simulink model "Noa_Nofusion_angle"  (R2020b)
settings: Solver=FixedStepDiscrete  StartTime=0.0  StopTime=Inf  FixedStep=0.01  RelTol=1e-3
PostLoadFcn:
  | if any(exist('dsrtsu_mdlpostloadfcn', 'file') ~= 0), dsrtsu_mdlpostloadfcn('Execute', bdroot); end
InitFcn:
  | , if any(exist('rtifpga_mdlclblib', 'file') ~= 0), rtifpga_mdlclblib('Init', bdroot); end,
  | , if any(exist('dsmpb_private', 'file') ~= 0), dsmpb_private('dsmpb_mdlclblib', 'Init', bdroot); end,
undefined symbols (not defined in the file): ACC_TimeGap_DecSetSwt, ACC_TimeGap_IncSetSwt, AccelPedalPosn, AccelPedalPosnVldty, AccelPedlPosnDiagc, AccPedalOverride, ACU_ShiftInProgress, ADAS_Posn_CurLane, AESSwtReq, ALC_SwtReq, BrkPedalSts, CC_ACC_CANCEL_OFFSwt, CC_ACC_CRUISE_OFFSwt, CC_ACC_DecSetSpd_SetSwt, CC_ACC_IncSetSpd_ResuSwt, CC_ACCSwtErr, CharSpd_ms, CSA_NODE, CURRENT_GEAR, CurrentGearValid, DiscIntNeverNeededParam, DrvDoorSts, DrvSBR, DrvTrqReqOvld, ECMACCInterface, ECMRespACC, ELKSwtReq, EngLimpHomeSts, EngSpd, EngState, EngState_PHEV, EngTrqMaxActSpd, EngTrqMinAct, EPS_DrvInpTrqVal_HighReslolution, EPS_FailSts, EPS_LKATorqOvrlDlvd, EPS_LKATorqOvrlDlvdVld, EPS_LKATrqOvlDlvdSts, EPS_SteerMod, EPS_TrqSnsrSts, EQ4_APPINFO, EQ4_LA_ELEM, EQ4_LA_HDR, EQ4_LAP_ELEM, EQ4_LAP_HDR, EQ4_LH_ELEM, EQ4_LH_HDR, EQ4_LRE_ELEM, EQ4_LRE_HDR, ESS_PedSwtReq, ESS_VehSwtReq, FFogLmpSts_F_Pbox, FLWheelDriveDirection, FLWheelSpd, FrntWiprSwtSts, FrntWshrSwtSts, FRWheelDriveDirection, FRWheelSpd, HazardLmpSwtSts, HCU_AccelPedalPosn_Diag ... (+151)
libraries: simulink x138, dsmpblib x33, canfdmsglib x10
(part 1 of 17)
PreSaveFcn:
  | , if any(exist('dsmpb_private', 'file') ~= 0), dsmpb_private('dsmpb_mdlclblib', 'PreSave', bdroot); end,
CloseFcn:
  | , if any(exist('dsmpb_private', 'file') ~= 0), dsmpb_private('dsmpb_mdlclblib', 'Close', bdroot); end,
settings Model: DataDictionary=HWA_DDs.sldd  RTICANMMDATA=struct('GeneralSetupData',struct('modelroot','D:\ADAS_Store\Project\adas_project','generalsettings',struct('filesettings',struct('destfolder',struct('Name','RTICANMM_FILES','Check',1),'buildfolder',struct('Name','.','Check',1),'AbsDestfolder',struct('Name','D:\ADAS_Store\Project\adas_project\RTICANMM_FILES'),'AbsBuildfolder',struct('Name','D:\ADAS_Store\Project\adas_project'))),'options',struct('addpaths',1,'rmpaths',1,'addtrcexclusion',false,'cannavigator',struct('checkmonitoring',0),'show_usrtrc',0,'use_usrtrc',0),'advanced',struct('options',ones(1,100)),'MPSetup',{{}},'RTI',struct('Type','DSRT','Ver','4.4','Date','02-Nov-2020'),'modelname','Noa_Nofusion_angle','block','Noa_Nofusion_angle'))  DSRTSU_INTERNAL_RTIFPGA=170  DSMPB_ID_DATA={'108889',struct('BlockId','81ba8c02-39a0-4bf8-971e-fc8bc9e1d8b0','SignalIds',{{'e6dae809-112a-4cbc-98f9-354c12187ac1','31d2deb7-ef93-4695-993d-314bc5bcc843','62343d78-d15a-4a45-8693-ba2849e89479','c13156af-d15b-4771-8a29-b8e73d565fa8','cbe04a47-fa20-4770-9bbd-4a07b568eb2e','59e00f7c-c03d-4b80-a5ec-a7b536bc6272','3f246c43-0baf-4388-bea8-c24249e8d124','05e7c6b4-9822-4e1b-91fa-c2d47c80a9dc','3c91b297-0034-4136-9460-a9a71fb1b160','b0eda23f-b1b7-44f7-9430-f2199b0de4f6','d9349f60-73fd-4e07-90cc-b8a5cfade7d1','f893d12f-c8e5-49d5-ab09-89fc2cdbf4b7','b489956b-9fe5-4db2-8485-d07366cb4569','0fd99c70-4fef-4ffb-8340-8501f6b1f5e4','53dd6ff7-6c1a-46a1-9139-61ea4f9d24e0','93fe1b5e-8abc-49f2-ae51-04c114465812','9444d888-9a75-4226-ace5-9b052183c8c8','ce7a08f7-cc95-444b-9a6f-cd5054dc142c','683a3bb5-05b9-4d71-b570-d34d769ae407','6e290ea9-9348-4509-bbba-48e715a1ad64','385761be-a1f9-4d98-b926-1efaecbe94cf','77479779-8c39-4f5c-be4f-4246b8ca51ff','094c4e00-d8db-4561-82fa-1990a2a46c70','8fedcf21-59e1-4a11-b24b-5edc3eea11e5','de2ede37-26b1-45c0-988c-7281b852313f','ed4cfff0-74cb-4a5b-9058-099c9444dc97','d8a92eb8-77b2-47c6-a14b-19e5a6c1880a','bb80831f-ec06-46fe-9a60-525cce3db11c','089a9e8f-4e14-4d97-a75c-e18256b8f73e','116e4020-4c03-4eaa-a133-5105e1ad6c2c','5d390f2c-fbfa-4acc-8e45-8a78ede6d630','e0ea540d-a3ce-47e8-9630-4c2a7c2611e9','1338e80f-eb11-478f-b148-febac8b5f561','40cb9f5e-abe1-4c5a-91b1-6a21a87629f0','f68eb2ae-9d65-4ce4-8ae6-7911307f53aa','90ccc115-d294-448b-be51-2f0d4ed4df75','d061fb9a-9168-48d0-bfc4-e7fc980285e5','66fbeac1-5405-448b-aaf2-b3b4c802c6b3','18d32c7d-1106-4865-b268-b9839028e3ed','68ea3199-eee5-4804-a61b-b9492c15cc17','251bf7c6-0b5c-4442-bed5-124eaca4f0a3','5c44ff7b-7cde-47e3-997c-d7e4d571a688','a318a3ac-fb11-4e42-abce-b283a20da434','8ac8bf9e-cc00-4453-b1d3-1d8cb9e4d5f3','e889ec5a-b6bf-4115-bfb4-789ddcbb1b39','843277e1-c8e1-4956-bb5f-69810b3fca13','8015402b-cae2-47f5-b799-3258863f20da','967f47db-98cb-4b9d-8737-8d02120e8039','408e6371-4b24-4e9e-8575-3f5fd9116599','0add38a7-641b-41d0-9036-40ff81d44c7c','42c9e777-d5c1-4821-b220-ee42a71da039','1eccc895-bd9f-4c89-9169-915b3accee5d','c32a22ec-25cc-4381-9457-3401f3ef52f2','dadafd58-4047-4fbe-8c61-d0d4f2e948e4','33df5bd2-20b0-4ead-bd24-c6cd609c4787','a6ef951d-803f-431b-afeb-b8db87ab93f4','3d89e518-12b9-4d0d-90f2-936f61a4e4f2','f4fba2eb-28a8-4b3f-a3d3-e6a85bead6df','1bbb28d7-2fef-43d6-b55d-c5356e90e304','46c1d4d9-bf71-419d-bdfe-9c3255f570d2'}}),'112056',struct('BlockId','6913c789-035b-4c0b-bbc8-df30b7210019','SignalIds',{{'6e67b619-d0e1-4489-8e12-cbb641b6930f'}}),'112939',struct('BlockId','bd32a928-034f-4d93-abe8-55cc1037974b','SignalIds',{{'ed378323-8937-4e58-90a7-af861033d965'}}),'112945',struct('BlockId','c5ed9ac9-a557-4e9e-b1b2-178e2ab00d3a','SignalIds',{{'9bf7ab65-611a-4ce6-8553-94d5ebac5e02','125861c6-7b90-4e8d-a590-5d6d82b8a9a7','4aee84b7-a55c-4fa5-a4b0-5c93a3e16834','bd31e0e7-f9ed-4a3b-9100-c48940e83979','f56bb652-89fc-4dda-9d9a-1212207cf3a7','0e2341be-0c6f-46b5-93e3-ba9acd4843ed','91d7f4b2-8cda-4163-9f74-f5dfcbc91f25','b0e338de-3225-4d50-a22b-4e417233ad31'}}),'21535',struct('BlockId','2585067a-bea5-4000-9f4a-5d4a5318ba82','SignalIds',{{'61f4e782-3c5c-4d26-b38e-7ab3a332c17d'}}),'21547',struct('BlockId','85c6324c-04f2-4bb9-ae49-a2215b872cec','SignalIds',{{'0e3885c9-c264-45e6-aecd-762fe1b73c31','1baabd13-ee21-4652-b6d4-ec6abbd58849','7652d1e7-3cbe-41d8-a4c1-1dd8e2fc5cb9','7bbccffc-d9cf-471f-ab9a-2a8c4994da51','a802a3dd-5a68-49d5-873f-4e8d27fb760e'}}),'26900',struct('BlockId','c4f53095-7434-4139-be7d-a6809331959f','SignalIds',{{'daa0d7ec-f8c9-46fb-8b57-637f6db1364b','6b9c406c-00c5-4598-bbc7-09f21b6102e2','f500b1a5-0ce1-46bf-9e31-2456a376294c','36025600-2dac-46a1-aa45-8494d12b2b41','ef53cc46-8ba2-4a58-bf53-0f87942fb3de','aa030106-e465-4c79-b00e-eff259d242dd','78eea2a2-72c6-4500-b175-67cd22d16487','1c2bede2-8500-4539-b1cb-e0ab955ea810','10a968e6-fd01-446e-bfca-b73896cbeda6','89b054e4-6567-474a-a101-bb566c01b012','298b31ac-930b-4ec4-925d-86f99e03a871','2a5dd987-b795-4b42-98e4-8e4e541ea47a','183af005-0028-4aae-8a97-0fded965b013','e1c3b11f-1e55-421d-b1c5-035f3444791f','d773bac5-9a48-4d62-be27-c6d96c81982f','04b9c5af-52d6-4c58-9c78-c1c20705dd99','e1e41399-89af-461d-9139-724a4d7cf416','0d5a1764-fbd7-4c90-8796-3b694c1b6f3d','99595cc9-51a9-4762-9eaa-0287cd22b3d1','74982970-242a-459f-a626-09b1e996aab8','e671e317-8ad6-460f-a115-14bde9303d0e','6aba3e83-cce1-4f14-959f-1b3259b2219c','3c1f9a12-89aa-43c9-9263-ad736254725b','e9e09c38-1a3c-4db0-b8eb-afc41c15f7ae','7d67eb52-960f-4419-a7b8-b5b57287a7ce','13d4f68a-7df0-4cd5-96cd-74a942b01dfb','b6834f02-cf2e-4d0c-83e8-3f5fbd5b4e80','11661590-7352-4bab-a498-0526255a2208','7f683842-0121-44e1-ac4c-b8ee6cdd73dc','13607d16-4de6-4b14-8b9a-e3fa31395056','9d7b37ef-0bbc-4717-993d-2cf555115b85','9cdb844a-f57f-45fa-9e48-b4a1a4b4896b','d36d0705-fbbd-4a92-912d-3076a1fef339','f1064f2a-d7e9-4f1e-a640-9b2d88534320','c7acaad8-e629-4dc2-8e05-0c6a9ba8cd34','12523044-5a8d-4a8b-aff1-248d7e37c730','d6a98294-c583-489b-9ba8-57c74dc9e44b','a662749b-cb79-4e22-b746-fb2c743a06c1','f430f874-81df-464f-a7d3-30981e4f10a2','beebc79e-c796-4a43-8cae-d93d3757c9ef','45edb788-142d-4d5e-b6bb-3d5a239307d1','f11dc556-f569-4261-bd02-c87d51a35c06','9fdd9cc9-7219-4342-b284-af726a522230','30d94524-5be1-4cf4-ae3c-2fca7636de21','0a9cc0a3-0bac-4d2d-8fdd-7eaacc91cba7','515fd30d-b8a5-4bf9-afb8-efc29c139c1c','7e6ceb3c-7950-428d-ac4b-43dfc5d8e62a','9a0a1488-4d4f-4ee5-9c00-712f8d888565','437104cc-392f-443f-b249-3988251c6d1d','ffdcc33a-9507-4d93-b2af-a5bcbf332fcd','ec49087a-871e-417b-9f51-df684f8a506d','9c70bacf-569a-4b32-9a53-2a08a50f21e1','c02297f7-a9d1-4ad2-9a5e-4508cee9802d'}}),'27021',struct('BlockId','bdf40dee-effa-4f83-9fca-9a80da5144bc','SignalIds',{{'6c1ed526-1be2-4bbd-bcae-90132b9ce65e'}}),'92096',struct('BlockId','2626a49c-eafb-489e-9e25-3cc30e7f0f4b','SignalIds',{{'3d8ff92d-3a53-4791-a9fe-7d0ec83fe68b','57fe1359-b477-4052-8b42-8fea101ccbbe','7ab6ec8e-bb47-446d-9b63-efa3400f4bc0','aae3fe2c-9486-44ef-a174-ff35666d1ac3','2728f40e-e3bc-46dd-820c-09fc547a2cf4','97772696-4328-4ad9-a419-0b1a5b3b5793','ee295b70-1271-4646-9bfa-8df6089991a4','624522df-0b73-4097-be1b-483fbaec0508','da88715c-b735-4415-8099-7b8d0dbc153e','ff209cfc-a262-4f28-baaf-3a6db897a966','e492b0bd-e407-499e-a6ad-460a06daea81','24f4850d-92b1-412a-9afe-0ffa2b28ac6e','e62d0e3a-07cf-4f2f-aed5-4364b9f58ffd','a952210a-42a9-4b58-aa64-8d3d5d349e0f','4a7d5fb8-0f46-4176-813b-55afe5653e46','44439239-e225-44a6-ba08-400a080bd9d0','d9d40cf9-f368-4b60-a6a2-4bed2dde0f48','50613ba6-c87d-4614-bf70-f0dff690fed6','171e7712-0418-4998-90fb-cbbc9f6a25a3','d8d9e3e9-d156-4676-ae37-3284503a7c6f','70f23cb8-d3ac-430b-8269-5a073a7d408e','efe9449e-e772-485f-b06b-2486dfc19974','7c476018-eb97-49c3-a1cf-2bcf515b1ac0','8ec107d4-18de-481c-b547-a0727ab809a5','45accd66-167c-4db8-ab27-6523ea2eac45','02953ce1-6202-4abb-9238-8ced4a0d88da','dab9925b-7344-4ce9-8745-111b6e6cae7d','c76755d9-df78-4ade-a507-373d8308233f','5fe272f0-e37e-4cdb-be86-e2af3525fe24','5793162b-b485-4d01-a81d-f3a4bacb08e6','a8a40964-43cd-4989-95ed-855ea1943846','f7248f97-efe7-4f34-b16b-ac2ba47ee6ba','84c9528d-5a3d-46b5-954d-d578c4df8378','3524f1a0-9033-4392-b170-0db3a27e414e','b9c5b901-2ee0-4cc1-a573-c8f9972649a5','b8ef879d-b046-4200-9baa-8e8fcd89cfbb','20f476a7-cf03-4f2c-a2fb-85aa3b4d50a6','caf3ad97-2086-496d-aaf6-47e61d3c29b6','c7efd7b8-2c78-44da-ae3a-28429611f8dc','45aa4b4f-2eb9-4971-82dc-61f3e357c005','2ca95a23-55a3-463e-975c-13578ef7d1bd','62c9d3f0-5102-4467-8adf-cf0fe7aa516d','e686d2ad-bd77-4dc9-b165-65d6d19e2eb2','9f4da501-daf3-4c3b-98bb-e7c10ddff144','1f52e3ff-314d-4fd2-9f3b-2179e824ba31','2af83930-d728-441e-9e4f-34537c4a20f5','e8860b5b-8674-401b-b995-34d5e2206f38','9dc95bcf-a38c-46f4-ad2d-2620ccd6e28c','b11c0df1-c523-4f91-8153-b13c114b944a','8b19ff0c-f7e1-4ee8-9507-7bfef01e81b7','e8150809-c884-401c-91ca-691eab8713b8','67b8761a-57df-4479-a70d-848ee2300e71','e9f52eab-a319-400d-b795-24d107b9bb7f','b66e22d5-841c-424d-ab80-4f02e6ec04c3','3d9b6ecb-ddee-4913-9e3b-4244499aa60e','593c337f-f38d-4a78-add4-e57c457ea88a','fdb5510f-5603-4091-94d5-66791780d419','9911966d-5645-473e-80de-5d7e0f980f21','6f7c21f8-8e7d-4b72-bbc3-0e10cb05173c','3cf030b9-a9fc-4f36-b3cd-b0ea10075552','5e21e0e9-e6af-401b-b8dc-f153ff7859a5','2ead1bcd-f571-40d5-b1b7-984cf6275c5e','676f31e3-b6c7-47a0-ad43-b760f2ef7778','366bc5b9-34ae-4f7a-b39d-9bc22bff78ee','550b7788-b500-4a37-bf74-1cd332e45fca','ed532467-088f-4cc3-b99c-2be22cd1f55b','5fe4a452-4c8f-498c-9e74-056d5e5fcb6d','de61477b-8899-4695-931e-e6dc9dff6f17','f08850ad-85e6-45a2-8f86-9c970bf65da7','a50dc5a8-222d-4853-a56b-c4c5f2030a28','1e12c040-3fae-4e1f-b57c-aed15b50cb60','33b8c258-adac-4232-a5aa-7cbd27f89e64','30c60cb9-0158-4875-b17e-2201775d3ef4','0158b5ae-3f92-4d64-a3ad-bb7474bb3a6e','e690eac3-fa9c-4927-b989-add4c8060ad0','af05ab49-1078-4638-8a14-6509f6efd732','bf24c6f7-dce4-4516-aad7-4a8c032ae8af','81991912-ea4d-4e27-8e78-5b0c76654bbc','c7fb6541-eaf8-43b3-b2ca-d9d981ac7d0f','58b9113d-cd63-4934-97dc-b52c923767b2','96e7cb82-855f-4587-9d3a-d7c5bb8fee74','c554e833-9797-47e7-bf0e-8b9fad210e74','cd4d30c3-fee1-4580-82e8-4f0beb8ab679','5834d1fe-a2db-47bb-acf7-aaea5892158e','7cf871d0-24ee-4dd7-9c90-16f120070cdf','7dffb819-f00d-4891-8820-5398d5acf060','24b69ebc-7c8a-4c7f-a3a9-5e9f7c52673e','f2ec1d12-c3d8-4df9-9d1f-8c9d9cc284f2','5ab44027-dfa8-4291-8ee7-384f014795d5','0c446405-c1fb-45ec-8845-28063d3c79cc','01d340e6-0f15-4ad2-8525-35bf2aa956dd','204515fc-fbea-4f63-b894-eef527e6bd9d','e0dca325-cb84-4f09-b568-622b6d4ccf91','60797110-5ba2-41dd-9826-79bd67f11f65','6c59198a-d826-4935-9238-c719cd5105ec','5f61e17f-4507-42cd-aa76-6f1039e0b56f','590781bd-a45d-47f7-ac2d-8a76d193c4ca','06b5c281-2053-4949-b9c9-acb1373d506c','829bc97f-26da-4467-981e-44e81b1cf974','d244fbcc-aa84-45b9-a934-2d34beee6c10','c03a08f6-16fb-43b3-b945-8ea80b9c454a','78b58307-773d-4ad4-ac80-3c426eb6d4a8','25944f9f-e7bf-43f5-9f90-4698741facbf','d139a39e-d189-4e55-94a8-a2d8b1aa8d57','a22eff47-2099-483b-bba2-0f2b5f9cd86b','1590cad8-88cd-4028-af3c-d2f3d779d367','86f8be12-a4b9-4ecf-87fe-8b25adef1b13','44ad9a06-49ee-4a33-bb9a-53a876073052','544623b1-218d-4bef-9f32-24cd6382c500','56dd516b-8b28-49da-84e3-05e53df87f53','fbba60d8-75ce-4bba-a6b7-394aab10a38c','536ac807-a0ee-4cf9-8faa-3ea45ddef2f1','78655c66-d146-4cad-97de-3e0ecdd3a2f9','db33c394-c73b-4406-b43b-5dac604c1e78','28e623dc-2b5a-4d50-a8a2-c5277908705e','85751a1c-63bf-4f97-9d1f-adab5e2a19a8','810aac47-5472-4f25-b9e7-f9f905304e89','18687fb3-d36e-4bf4-8873-298926c4bbb6','68c8c97a-1822-40b1-813a-27642dfa48f1','48e55f21-58ec-45a9-b6f1-31ef51cd1bf0','4cc1ecec-4a9d-4339-8d09-837ffcc25a27','0eaf747f-be20-4679-8033-16d430a74668','71f1aad6-0a58-4bc9-97cf-f58e1d8a4d7a','a575f744-505c-46da-8164-3f27d1a01f29','88c346a3-1222-412d-8c82-18bb32cb94f6','9c4dda8e-2c36-4a68-a520-345222c759f8','9a64fe60-86ec-4c53-a8be-0c368dad4863','cb05c1d9-09d9-4691-be10-38ccfdb68f67','20a3bf7a-1982-4296-8e2d-403a73f32733','eb52f21b-ee1b-4288-a0f4-332dcf652d5e','f65cee83-56b8-45cb-8458-d0096cf4994e','bab032c3-1da4-4612-9dc5-aff2ca75e79d','5176ddc3-9445-4ad6-a31e-042e42e290e3','d10d9d92-94a2-4b5b-80b8-f11cd38c3a59','5691495f-3af5-4ca8-844a-29a1f4400004','7c53693e-f3f0-4fe8-a3a1-54ddaec8b4d9','fc96d5ff-d377-4bbf-a28e-3e6a6dea7dd5','1e98929b-e7af-476e-af77-181ade8e652a','db202cee-d525-49ce-a926-71f25cecfae0','f23ee0e6-90c4-4426-bba6-88df4a770310','27e0d418-cfbc-4f53-ad0d-eb138646fc32','e585dbd5-ed73-471e-b9f0-10ab4a80ee54','07204a56-ebfc-4e5b-9c6d-82f4c0129d6e','90822bc5-41f0-4928-ab6d-fac63b5813cc','46c69ce7-cc6e-49b3-ae8a-a82c548a48ef','7b6ffa78-10e5-4210-8134-880aa24d68f3','94c28e1c-015a-4654-92a5-445b6d750e09','fee0eecf-773e-4070-a917-a579c9a22070','35c0ef53-0794-4280-a40f-615abcf31fe1','2e7a2d6f-cc05-4e9e-b974-61ed38c5e3a2','c8a5d024-bc45-4303-aad5-443d5a088151','531f8683-421d-4c50-ac9d-75407f48093f','f5b45fea-f8e6-42cd-acd6-91eb016667d7','28910d08-4039-4b9c-8464-6b26316e2112','a2e4e76d-37b2-4ee5-89cb-2016e27c3a0f','e25a7e01-8980-419f-984a-184cbdcc3045','7caf7c64-cfc6-4577-91b2-7b0ae61a5b70','f14a134e-e223-41bb-8b67-368551a07fe6','850e7f72-971e-48f6-b743-5f389edc33f1','be231029-9743-4673-9108-ade630e37c12','e2c6fd4c-3723-40fd-80ef-771b8340b045','0419d3dd-643a-476c-a243-f1eaa6a780c3','a683725e-482b-405c-a89e-a97d565a6064','8a4e4ce0-eaf0-428d-bfb5-d3362f879d15','e8b44cc4-137f-4451-aa6c-b51e1d43f117','000c1bba-a30d-40c8-bbd1-d305027f6501','043d9aa3-06c5-4059-9f63-2f6a5b7f1351','3f1e1b05-cd4a-4187-be4a-bf0ed78c3c42','d5757a81-b479-4372-a289-125bab7eb450','a3fe406d-cafc-4714-bb45-dc188105481e','38c6a662-de1c-4f75-ba1f-03d816189bb2','9b388ea7-b241-4201-85d4-239a0b36b8b7','8447252c-5f40-42d8-97e7-58ce273fbb3b','afca203f-fb32-4c43-9256-651048cb904e','04418faa-346d-42e0-ba90-20a3a68eb760','2e4f26b9-fbb0-4565-b220-ef4bd4876878','3f5e17f8-1d4c-466f-9a78-91929891ff2a','84465d9b-1101-4a34-8139-fab9fc9cbf4f','0de2d0bf-9fa0-44d2-893c-bcb712810756','dff52e5c-f10c-4e45-aaee-e871f06641fb','f58df008-19df-4468-a02f-efcf04c20781','83fb9323-d1b9-4495-95e4-c27cc9781ecc','aa7a6970-ca01-473f-8a65-a664dd364882','15332edd-13b6-4e95-b55f-1ddf2e4310b3','349fbd14-9300-4ff8-828a-1d78de258286','d0fa0445-40a4-472a-8913-8ffe2b60f13d','ff00bbce-7e63-416b-9fdb-4ed606b1a647','5023b9ad-1d78-4877-8621-66c99cbf9033','831d24a3-d149-43f8-9d5b-5402989fb5bd','805c8c6e-14d4-4dec-ad85-2314cb821987','5eb82689-b93b-4494-86b4-5d80ab075d18','122caa9c-802e-4351-a0a9-ed314f74f62d','b758e3da-1b08-4627-95d8-4267f30be063','9a29bf84-d57e-43eb-b40e-d47ffb77341f','1d1dac37-4d36-47c7-9661-96a4fdedacdb','2f29f70b-9b09-4c4c-974d-0d5004e34c80','642c19cd-43be-482c-a9a4-a822b4bcee85','e1288f9c-444a-4c82-832c-12df2471b08d','4587c4ce-f20f-4063-b6cb-58b15651d415','20fe301b-8a8c-4ea5-9763-048fe2f63d67','050947ac-02b2-4c95-99c6-1ab11244084a','93fab8b6-c071-4a2f-bb64-4a0ccf61c80e','fa2d3185-53d3-4297-a3a0-a5a26bba4129','41f55103-b8d9-4268-9f4b-38a1c7a2e090','9131575f-1513-44c4-8e40-dcea1bdc2c34','0f6f99df-f496-4d71-89d5-9d3f90c03f66','0784ce9a-c36a-4a5a-8079-f53b5037dea5','dce24de1-3b73-42a1-8d7d-b9ccc29b5585','613e1a0c-6586-4f78-abf8-e712a4506a21','325f16a7-6461-4dd7-bcfa-d3307cc77cc0','a56cdef0-1577-4bbe-a286-9e472b92f1e2','69fe0482-a70a-45cb-abe6-38f6e9ce5682','a1349f06-44e3-4a56-bc28-57c886e1179a','b17595e0-ef28-4479-9f5d-200244451920','90e25904-45eb-47b6-9092-c7ea319011f0','7a69f69e-ad38-4652-a990-2f14a164b033','830bdcf8-6bb9-462f-ae29-93ef8a59ba0e','2c0f0daf-9967-4453-994b-4ac2b76a3fe9','f86d2f2b-5748-4976-9625-ab8d5fc01a44','c4d4b03f-4b49-4fd9-bfda-5580df38df97','805d6294-3f53-4ed7-beea-f7762331b702','1cdf3370-4712-4d44-af91-44d4946fa4da','8194d2ec-5f1e-48e1-b65f-28fc37a23c0a','fb58e5b8-5237-4940-88b2-272d03922783','ad6c4650-8134-4838-add4-c8bc474b4668','72eca40f-2206-4b85-8624-1b6ae42f537c','044e3b49-78a0-42cb-984c-e66dcd598d05','8efee970-1d6e-414c-8f03-27a1d76d5a0f','97d41cbb-8d5a-4a83-9ba7-185b7fe2ea08','d68f95fd-b8bf-4d01-af7a-b4fb6eaf29c2','303db2e9-fc92-48d7-9ecb-906f70e1f416','eed1e3b2-fe0c-4562-8b46-54d63f8a7be2','651a94c2-122d-43a0-8367-ba20cb93991a','aec85a4f-512d-4291-b810-978491f2380d','a1ec1e82-f988-4698-b178-4f40f74e89dd','24a65454-a01f-4027-9898-08fd81dc5b4c','9e32fb24-0ee1-4893-ab7e-c2ed85e083fa','0ef10c6e-1151-4395-8f2b-6039b664dddd','3a73158e-3018-4153-8ced-d8d0e52f7920','17cd7138-e8bd-4f08-a03f-4a6c28dd26b3','dc6fe649-0f9d-4473-a4cc-c67f096792bd','3ff2c654-08e6-4a2e-a2c0-f2ccca39bd9a','267fdbc9-0013-4378-abac-1a3bc2508325','8cdcbb97-c6af-44f5-a81a-fca93d548d85','01e47132-7cb7-4a8d-b3b9-4acb1b5ba713','8adc715e-501f-43e3-b0c0-daecd1c071a4','f0e897b1-8dba-478b-bea5-a1c344bcc182','5dcf6f94-8217-4b56-b241-d3a06ba668a1','548dc5fa-44b2-4cdc-8253-6ed94beb141f','9518475d-e0f2-43f1-9d95-d8dd24590394','0a818e29-04c3-4567-bc47-310dcaf3d1a6','4308728a-b992-47f6-8bc9-b6e3f15d305c','1c3d6196-d166-4677-9203-c0a470623360','593a4882-3d5b-49e9-913a-e4ae0053ed37','d041851e-159e-4808-8d9d-19afdea47f88','4e06a3b3-ac88-4829-8269-0227281a727c','fe6471fc-70f9-486a-bf1f-77fec6457f9e','99d3fa79-1be3-4227-bd24-6e9746d4143f','a242adca-2b2d-4c38-8b84-0e9f4200f46f','e0312b30-d87b-4033-8dc5-803a5afeea56','e0b2bf1f-6a31-446e-9a38-87510d2ee6d6','f3d1dad0-76bd-484a-9865-5d8a0acf70ed','90a56866-adad-483f-a6ba-78f4b2b96364','6ef1b725-24c5-45c2-97f7-e06ae2b54272','7ca65932-c1cc-4218-8b36-982bfce690ef','0abdaaa0-732c-4bad-97a5-d541d143fd51','4580bbaf-11f5-4cc3-bdc7-6ba801093fbc','ae10fa7c-a526-46f6-bc3e-748a89a638fb','52432646-2d18-4636-a478-5f06272abf7c','58e81fc3-1290-4d08-83f8-c00e55bc61a6','c00e220c-50ab-4f97-b452-eb2acb0b0a38','4172b606-5824-4d39-9648-2c7e0c22fb24','92d5bc23-8f61-4ccd-8057-7934b5207acb','b948222e-6ed8-420e-bd4e-ccdcab12feb6','fa6d2daa-a272-414e-a20e-acc675712022','9dea2d2d-8814-4ccc-bcae-b111e1d9e5aa','54a8cf29-9aff-4017-8f9e-428b696d1089','87f29953-f87c-4770-9e8d-b92682e69ee7','cd4429c2-46d8-460a-b491-30d9c09fc7e4','992b789f-633a-4c0a-af80-5b9957a64f4d','cd96e18c-3161-4947-923f-704f1673541e','462109fa-53f9-4130-97fa-2cdfcf16764e','53aa0027-9c38-44e2-9ff8-11d8417f8f40','ac09190a-e396-4807-9600-d9fc98987922','965915a3-49fe-4e02-ad50-727e3e372404','2ec764b5-b421-4acd-9aac-9a2d38a7756c','61309634-1525-41ac-b1e2-f3cd920aba8f','d9bedbfc-3228-44ec-bc52-2f20e8a4efef','7a3d64b4-ec3a-49a4-b5f7-080940d90220','bbd22767-c34a-4a65-bb76-b8380c69f21d','ad79eb07-af72-409e-bbb0-85bc82707581','5c1507c2-9c52-43e6-b66a-79c718379997','c0331f0e-3149-47a5-9c34-c7d018c92a10','8f2db1ba-a0c7-4209-b52f-8eccad69a858','84c6bedc-52c7-42a1-a0a1-b4a7542e9ed9','1f92b609-3585-4b61-b2db-778546bf6a8e','01d30e4f-cac8-4824-93af-2c1aac36bbee','1c89c759-8a54-4581-95ef-e26b3a733658','ee674abd-2a37-4259-9eb6-d9255888ef59','f7fd4cc2-8d76-486d-930a-33f5615b083c','dba21ca1-4bdf-4256-93a4-396ed9567692','08368ec1-99dc-4993-b504-6e534f95d426','f7c68234-5b90-495a-b707-1e65d1a8d37f','d1a3221f-32cd-4871-a58d-8f09c41f27f5','0112242c-0417-4ad5-b3c5-3a459f843b2f','1e04c133-d319-482b-9251-df40ea67b952','e3caa92a-8aff-4969-9a66-8be756e416b3','bff3988c-0f04-4c00-ab11-511fd2885bf3','eb697231-e7c2-4f0b-8d08-3e2dd3b4bc61','da7f149a-3bbc-485f-bd77-e8024b9ac6b5','1970c710-01b7-4869-b3e0-1e5614a42f80','0e4a3b2e-da26-4b6a-8a04-f0448d43dee5','2090db71-2e79-416a-84c7-84fa5edd820c','fbacf9d5-caaa-4636-8d61-3c4aae20c5a0','0b794907-2465-4a16-96ce-03a3661d0a4c','5cf6edbc-c458-4222-adbb-ab36ab37922f','898d3560-a168-4d57-8ac5-9a1b49d5fae9','12e577df-4cf7-409d-90ca-61f8b3b69628','bbeff121-ebcb-4857-baee-cb9df93a1440','8f5c9992-fa36-47b8-904c-3c94a866fc5d','d3a1621a-0840-4db2-a6a9-d52c32742f95','044da422-aaa4-41ac-912a-a3ecf9bc9e93','2e0d1720-d393-4143-a3fb-dffdd518f6e2','94f19e2c-045a-45ae-9028-0bef41785d82','6d2e69e8-ae80-431c-a1c7-5a3af749dfb2','b13f59ab-a9ef-4c45-8096-a05a1ba1529e','baf016bd-eabf-4cf5-9623-d2492a80ffe0','0402e472-2211-40e9-83b8-81f64b39a834','1c0669c5-6fcf-4aa4-995e-ee01de78ffaf','76ffe772-3164-4a14-82e8-01cb3e790ec0','66eafd35-c5a1-49c7-b27e-01f2742a6223','151e4f6b-af5e-48fb-b8c5-8d7e1c4d16e8','9ea734bc-2b42-48b6-bda6-4ee1e2c507a1','c43f4775-bfb4-44c7-99be-d8ae236b5fab','a5544eb4-9c5d-42bf-88b4-f3a8071c5f34','cbc81f1e-cc95-4993-a44f-b717fdca880d','6e780ba0-987f-4908-bc50-38a8338ba23a','2947cd37-7e3e-4b83-aa29-ebfadc627cd2','f0d78749-ec35-4fef-998e-a36372f4242f','19c1c3b9-9704-45dc-9ecf-153593b768af','9f4f3150-dce1-4cdc-a791-d27b79529b7c','ae2add4a-81b5-4ef5-98f5-458fa7c1dd7d','5551d896-095c-4cb8-8d58-f3cb1761b068','3f7f7b9a-0573-426d-823e-001a842fce79','e95db9d7-7856-4ebd-9a78-0010bfd540d9','fc8ca16c-c780-42a8-b649-447d66deff20','a8fd2a99-d6bc-4412-8ba1-d94bfa2126a0','e1a70efa-db41-4cfd-b40c-c01cf48262fe','728a0f41-4209-4dd0-b562-cf253b8fce54','bdd9150e-61ee-4bc6-8b3e-43c3253b1aab','f5a24cc0-9cfb-4fae-8fe2-74074a21b079','c6bce8fa-674d-4198-8f60-d6969c79a83a','f21c9b29-6525-48fb-9ecc-3680e67cd314','597c418f-3f02-46f2-930d-2eb9c8807c97','8307be91-76c8-4d78-b268-e765f17f8213','b296ac75-36a7-416d-8475-ffbe6e28dccd','894d960e-802e-4f7a-8988-49627d5ba1df','a63e3140-6046-42d5-8e51-0dd32a1f13b2','8b1e169e-5056-439a-bec1-36baa2e9bbe6','a4a3995f-113a-4dc4-b25a-be8bd1da7387','86db2c15-45a3-41bf-8c56-214272ed971f','381093e1-ab66-4e06-8fa4-4456f17711fd','076fb968-2186-4b91-ac30-2c432f9a9177','ab926246-8b0f-4aaa-9f36-675b3e24831c','1c642a3f-1918-46ff-ba78-fb9d552662c2','e2f89cdf-10b2-4393-96fc-de0fa61990cb','d6804f24-e5a9-4555-a6b1-6f9220e6faee','5b9b6444-8e5b-429a-ab3b-bd226f4f6762','00259496-7a4e-4736-88b0-c3b2f79e1a6c','ce5c8401-1f96-4f9f-aea1-45add305c888','4b72b3c2-128b-40ce-b5a5-e6203ab8306d','a6696863-16ac-41e6-bdf2-7a9e7e2f50c5','5579eb2c-854a-4fc6-b271-5eeb4e997a7e','1a658b2f-1574-49ce-b65a-4246003d54a0','74560410-1615-4c09-8363-96550de29c30','b0419aad-872c-4c24-add1-f2860d6fdcd9','e97708e4-c852-40a8-ae18-987509e18a13','8cff1538-1894-4d55-b669-06693e404479','b4ed3a7e-f2aa-40f9-b923-b562909472d0','c4175113-de5f-468b-be98-58087cc64d65','74c16fa2-c833-47bd-8b19-6877a026f3b7','5b0411c3-d5cb-4aef-a067-37da547447fe','61c5c432-b1c5-43ca-b42b-5d4e80c0df73','b1af5bfb-206e-4a56-8ec4-1474445a9bb0','f2af43f6-5b91-4976-9137-7ac836e13615','8c65d3c4-3cc0-42b7-a4fc-d34618147aae','bbeb1f63-8ec8-4a7a-aa7f-0a0670ba8c53','5e0b7212-de20-4b90-8167-a1d8d71b3581','7d6161bf-e6c5-42d4-9fb0-c855bf3c35ef','c01509f7-092e-4f93-8686-3d0b2ee8030a','aada585b-6d20-4d9d-b905-db9ebdcb35e9','7395536b-d0bd-403a-9077-1497efab2e29','8c2fee1d-b5f8-4c47-8b73-94a48fda8fa8','0c480f36-c97c-4ac8-a400-ee222e844362','16a2cd31-dec7-480d-8797-555f0d0a5951','f4a70afd-024d-4f0f-b108-98c72aefbd06','26a6634a-5557-42e2-951f-9ea525d513f6','3f0257f4-823e-42fc-ba1c-f70d652cdf0a','073b2b0e-cf48-45bc-bede-14afe0caa544','579a02fb-b4f5-4474-baa3-be64164def26','b0704ab8-8b9b-4f88-9a9b-873252207f84','9fb165fc-676b-47e8-9f44-531aeddf420c','12021c71-200f-432f-b9fd-2e69e6219535','1d7c976c-cdd2-4f7c-bad9-d2915e0485a7','f042261a-1bbc-4244-a964-2c8a0400aee3','5d1e84a2-3a42-48b8-a30b-c4b129cb754d','d2d41370-9876-4a7a-8de8-82f700e2f03c','90c2780e-80ef-4d54-98c7-24cdec16d72d','1aaa07be-19a6-4a4e-b6c4-511fa69433da','29bff75d-aea4-44ef-8dc7-dc2cdad6fd2e','22ba7138-1ce2-4c61-a335-28ded396f934','989b80e4-704a-4c79-903d-8ae53082e8b2','fdd8c6be-3c96-487f-8664-c518a8233547','35bca300-b763-439b-b9bf-23b09aac20d7','2878a9f4-83bf-4f74-970d-26ffd3d1caa8','19b50e68-db39-410f-beea-1741deb1b001','356c795f-fb51-43fe-bbf9-7030ffa63985','fd17d122-5e4d-4f7e-a9c9-a6d311502c23','6f549206-f745-4fbe-bf4a-5971d91758a2','52b171e1-cd33-41cb-b377-677409a7428b','551f39ec-44be-49ae-99f7-8fbb47c7fdcb','d8292ad8-043d-4ab8-948d-47cfa9b3b904','5468b3eb-6bb6-4413-81f8-489f4a61756b','94faf67a-fd83-4b87-be96-f76b816bf144','091e0108-cdd1-4850-bd0f-da47856ad13f','419c7e64-d721-4347-816b-01c998daa6af','46a4906e-9ba3-4399-aa15-7a1930adf60c','b1daf8f4-29ea-4d18-b082-e664e9f00a9b','eca1e40b-03b0-4193-9add-170578cd8756','f85399d2-b264-4259-9e9f-004db37898b6','c3d31f73-a62b-4485-b7bd-52724527d350','be9a7d52-5fd9-4b4c-9cac-84dbc16e868a','280d8570-faab-43ae-8673-e4770aca2299','c2f14551-2fa6-4f5d-9652-86ed23f67bb1','654f0f09-1430-4fe4-92ec-50ce00b1dc5f','b49b834c-ec9c-436f-88fa-7366e4573437','58f0fadd-680b-4055-86a2-d55f3f3f8f82','51325ea2-6a32-4c67-bb76-21573a2169b9','bc1c4ecb-3aa4-4f43-8caf-4662ecbe2eb9','53d1839b-9066-4927-9676-63bbcad37348','d0060f5d-6577-4748-b4b3-c8b6ce68a578','3d0fcec5-b4f6-4c22-8482-8ff5ed200b59','0ef00a85-d4c5-40c8-8637-dcf3d4564715','5deaf227-9f03-4762-9848-fd8ef131a10e','dd0833b3-03b1-4a69-82f2-76d1e8bc892c','eeb776f6-7b81-4219-836e-3f3be3cd9695','20c66184-f6c2-4d0e-bee4-31bd34f6057d','d851385a-e66d-48b7-a8bf-76b0714d7a68','f1077060-e81c-48ff-b9e6-e70828d15019','fd80642c-b57a-463a-b181-2be25a097bf8','a9ebf9d5-2f80-42e4-8e20-38bb855c96e6','4687720e-f564-49a4-9c3e-f036b574187f','ad1ca5d7-4b96-4096-8c8c-67aaba8eeec6','50f88368-7cb7-4366-97f5-c5c325e90273','b7c92691-c7d9-43bc-b69d-92b843ea7158','60c03145-284e-4852-ad84-286e71e9ea72','e4dd28a8-995c-4fca-b0c2-ec4f24e2424a','aac9f0fe-ef3e-4826-b52e-c15681203e9e','aba80fca-825b-4c99-8963-dc1ee96d5b4b','2e45b1df-cd50-4b76-ab31-6a45cf9ae826','988e9de7-e2cc-4c9a-b1af-0357ac723711','3974ac48-9636-46cd-b33f-a733d462f3cb','0e4c31bc-9b88-4444-9e87-80ca52fb743b','c517967b-e221-44b9-9af4-12bd06773eb4','175e145a-8343-4bf6-94b7-9391521a5986','a95faa5c-3511-401d-b485-deefaeac2792','4b78abc4-2c5f-46e6-85ed-1c48369341fa','5e1f4c94-6e78-4788-b6f4-0ce9a3b99af9','73960f8c-ca68-4dbf-9e53-53729829fa51','79c4c0c3-359f-4fae-bd0f-703e728dc7f4','c5ef383c-7477-4fbf-8f2a-8c34570b0a60','879407c9-45b1-4cb9-a337-93d3db86b180','082194e7-ed30-4db5-8633-7802f160bb72','946af0f8-9335-4e78-80ea-1d5e85c38cf8','4e6f7f2c-433f-4c8b-b57e-0223170cef3f','1879369c-4975-47d8-b161-b9458b2e2e0a','bf825221-13e7-46b7-8d8a-6bcd9cc70f45','6f4aac89-67e5-403e-8ea2-3e64eaecf5bf','7596f3bb-92db-4460-93a5-624b2e104dfe','299678b6-461f-4c28-96e0-8124d01cf03e','010a117f-131f-4284-9371-9989545410a5','e4c22902-2650-48ac-ba80-c23785a87932','afd4b235-6a4f-455d-a240-409af2e6d646','8ad1ef57-2671-4903-8b6d-55e96aab5b8d','8bc62295-df99-48d3-8281-dca323b41dc1','5f3503e6-9146-416a-b65a-715c87891207','a978b935-72e1-4a6a-a353-e8e80c7b2e60','76243153-fd90-42e4-8b0e-49392d590d6e','2d324350-e7d4-4d02-9509-0c033d157d98','c4130826-e813-4553-9ff6-fd150077a4e9','bce17a2b-86a6-4113-ae93-9ba9592fea9a','2e372e71-df2a-418b-99b5-e60dcae02d7d','5705a4d0-231a-4f76-a718-743fc7760f97','426cfcf9-cd7f-4c69-ac15-b1ecddbf17a8','f36e64a7-5c89-4d76-9010-d827432252be','fd3acf14-20e9-47e3-8df3-591469caca75','0a706e06-c899-42c3-8046-58b2d3fc7d91','f5b1242a-cdb0-4af8-8de0-89eda9ee4d9d','bdbb7bd3-fcd5-4dc7-b094-8b43f8065cfa','4a2c0b2b-7407-41d5-b28a-9dd2e33d491a','aa7fbad8-96a5-483f-8977-f1ba9f15b5d2','160fa7db-1b26-438b-9987-cdbec0a93ad4','0763ba0f-efde-43e7-8255-56e978c1629b','6f4a8351-045e-4a29-a9ee-9b93daa006a4','22597645-6d42-4252-a7e3-185db38ec2d2','1f38a729-2f1a-44fd-b72d-137b48266fa6','e2f52da7-f5f0-4baf-895b-3029a291ce3c','8c543016-e72c-40f6-96a4-336a89459910','e6dbaa1b-97ef-4f0d-9256-b9810fe718b1','e1780a4c-0559-42c0-aad4-480aa5ff3778','4279d1c3-c688-4fce-a8d7-2ae62dc9ca96','2c8f4d07-16aa-4577-91ae-76df51f10279','5563937b-4b16-4ce6-b827-117152b4a5ec','1c991fa4-1549-4d78-8288-b10e4ca2998b','0b6d48e7-3820-4fad-88c1-63ec63443a08','ebe2e4e7-e2f0-41d5-aa89-f785ccc8ec3a','38ae271c-c8d5-4a03-8013-9ec2c47529cd','0790e15a-6b8a-4845-9d21-328a736df5b4','d67511eb-f783-4f61-88ae-1490d2572145','d3bdd845-64a0-46b0-b476-dca13ced2ffc','b736b726-8c68-48ef-b37f-962bee919652','b9a7c64b-9f8d-4190-9f24-e2f792e11502','10a527cf-1826-4f5f-b5a3-4ca107957394','ad926b5a-bf53-4a24-bb33-d2f9205e9bc0','eb285f61-3d8a-4fe0-b4d0-39bbbb443f82','c4ec9191-8bc3-450f-9716-6f453cdd812a','832f16bc-c43f-423a-97b6-e3dac3bffdfc','47583840-8eef-4d12-8cc8-76d2cb8740a9','bf1ab68a-13ee-4d90-b4ea-86e30b37bd0e','cf1292dc-e208-4343-b421-4cf754db4c2e','20886a61-9b04-49d5-a553-ac9d64afc746','c3af9811-6422-459f-bb1a-421cb00c9b40','1bafcaa1-913d-4539-b979-a7bfaa160706','70ba4110-ceb9-4379-96b4-bdeb2958aac1','d173cee8-057f-457d-a2d1-594155fd8c97','064de6be-eb39-47fe-a1f8-f9ba22ea3f1d','97a820a2-a516-400a-b99b-4f4e5ef57f5a','e42fd0d5-5d6b-42af-85b7-b1ca3c3c1cf3','1a322cd2-c4c3-4132-947c-faa7a3c08cef','66fcada6-8238-49ff-a455-05a7ac70b4b5','d719d213-e9d0-4e7d-890d-7236a66c7cb6','35af2bb3-a069-43f5-9803-a7d191e6351a','2f9c4c72-5013-4d06-8d87-ab23c5bfa9c2','96a21c38-6676-4766-a0e5-e08080a9520f','5296c869-810e-411b-bdb9-633e4e32eb1d','465b4fd9-9321-4312-ad14-8a1e8a50726d','59288a23-b56c-4cca-8e4f-f2065d3c487b','509e012e-2f53-467e-aa83-9f9cacc8d0ad','62b6f7e3-8f71-4782-a4bd-a65ba11ab121','5ca40bfa-1ae3-4734-9c53-2829ce432132','fd3b8df1-1bfe-499d-98c0-3955807cb63b','d5454e6d-6416-44b2-8fcd-45df03b641ae','eeba2715-54f2-4060-a6d4-22ac645c64ca','c330d381-3b1a-4c51-a559-7898e26e9350','ea06b3c2-401c-4c43-9465-899cf4b02a94','9dfd99d8-7703-4693-bde4-e9f628eef3f9','7d5d94be-0143-44f4-8429-4796c2bae2d8','1d298f66-a3f3-451a-8cf4-f6a3b8bc7073','20be5407-0a21-4624-b63f-9dcfa3be5014','9afb2d93-97bd-43a1-a71e-02bad8cc7d42','35b2b1ea-680c-4c6a-bff4-ecf48c461e3d','b5fd9966-9d0f-4834-afd0-682922e4f854','26713ce6-280c-42b1-9ddb-ab69fbaaf357','4a4abade-975c-42eb-9bca-5dfb163fdd80','017c90b9-25be-4655-a229-4a46f797dc86','0c081d88-2501-45c5-8eb8-5522f4a60928','61768533-6712-48b4-812e-c32fc1c1903c','613995a3-dc2d-4755-a168-c57b414ae623','35ac1f72-e361-47e1-811a-6f4af65cef14','c413fb1a-b519-4869-9bdd-356fc2e5b49d','533d6502-ecb9-4f8a-a641-250e2d300ea9','a7de0669-4697-483c-8121-812576ac89bb','986f277b-b5b6-4378-ae42-7253e0d752b3','bd096478-1b81-429c-9798-8898d0462079','2ffc8c68-6cea-498c-8772-59ff3893dfb2','4bcd4ca1-a484-44e7-8b74-ef661f99fbeb','2a1c9d0d-1e28-4852-a0f5-c845b846adbc','6ce1bbeb-6481-4a74-a434-22ce1cd42c96','f1e89aa4-fe51-4ea2-bbf0-fd2696ff0119','369acaf3-c8ab-420c-831c-d62d8e6f6add','2ab440d0-bede-4512-8641-c669afa8d779','3f9243bf-47e8-41cc-97f7-607236cb9ce0','7e94b644-3b66-4ac3-aabf-7efb9b02e982','f31605d7-bb3b-4d4d-a2e4-ad8f616e042f','162f003c-4e74-4914-8469-f0df090146db','866262b4-a6db-41f0-bf35-f112477bc810','ef198493-8682-429f-bfc0-6daf7dcef03f','4f0c6096-1f32-4d98-bc21-ee593552940a','12d27030-1fc7-4dd3-98cb-b4edd982143e','b8953893-d163-4f58-bcea-992c58a60294','26ce48e9-4fd2-4818-9f09-cf20db88422f','db9d6d98-7671-4ed4-8f6f-ae8284aecae7','a827bc49-aeac-4734-b7d7-ce386525c8e5','623ca0df-0da6-447a-af15-60e4af6d3c5b','fb4a2b9d-6024-4c61-81b0-4184b338b01c','50ce6120-b55b-4d3a-a7d4-1abc45dd00a4','eb150470-fafd-42ca-89ea-8e46a6f8da5c','fb1005d0-0f13-4d0d-aeb4-bac35f8ee173','d5f44f87-b192-4729-86da-e27b68a3720c','85130f6a-f200-420d-b5a5-2d5953bf8f7a','7c0157a6-a91a-4d91-8b5a-ad3951fc64a4','7a83f291-5dae-4ead-8e34-8b34ecb9de69','53a7088d-2008-4ddd-b590-0ed960c56c35','df62cd02-3f2e-4486-8d5e-cae5df3e5f59','6ec716c9-378c-46fe-8f65-74c44d7096a1','ca3632d2-f0dd-40a9-b0c6-c93e24d1bda4','2712b808-527a-4ad5-871b-a8e900c324d3','db275b30-f1b2-4d61-9632-369987df32ee','993deab9-9694-4b89-b3f5-7b8564f64ed1','909909db-0fe5-4311-b2d2-7ce40b22b982','d1a9d0ce-5a23-490a-a530-3374bd314cff','8b2c4a87-8afb-458b-89b7-4f47234e7dc4','13cc7f2d-e1a2-4481-88ae-1a05d1c4d725','5107f0d4-7763-493c-a242-99da9bd4f46a','70faa3f5-b3f8-48f6-91de-46baf564efe5','a956a2b0-2fa6-4ce4-82b7-63b9365052db','9a5fbd99-54be-4ce7-95af-0687fbb3e051','75f6fa05-56b1-45b1-84a4-2410aeabc8b2','455ff25d-9585-4568-b795-b248a58818fa','4566756b-2e5b-403c-8c46-37a81906081b','2333030a-30e8-4d8d-85e8-9fbc555ddd3d','1bec6521-9c86-48d8-987f-cd1745ee6b30','0351c5e3-1c8a-43cb-b8f6-e54e35b05c07','16187e80-4fb6-4e7b-8cb2-60af4c1391d2','c28a6d15-5ad1-4e65-8abd-ce3fa5a01623','8c8b01af-0dfb-431f-ac13-8594af838e92','30ac2d00-aef4-4f04-b780-0eaa33713348','91e00ea9-934f-426c-b017-c7b553ecc62f','5c9af031-37c9-4dd9-8842-c7b3c60dbae6','6d1a4f22-af0a-49d4-8d97-fc6fdcce42c4','fc611249-7895-4598-b6b2-76bb3eb1f39e','85da12a4-9498-47f4-b174-77b2d3df391f','e3b45f57-5001-404e-82b2-52d14712fc13','87d485e0-ba05-40ba-aeb3-88a566e8ba62','85c2090f-0468-4e09-8007-07adcf47bb1e','6515c45c-cc24-486a-a7f5-915f23d85d81','343bf17b-60b0-4d3a-9b46-58041e27c0f5','79a0cac4-8e58-45f0-8fa3-64d74cee8ccc','abbff1af-9246-41c4-b93a-7a997e0892db','9fcf36bb-beb8-45d9-b645-ea64cf788b94','e5fc7547-f296-4cab-9be5-0403fa932e98','28208496-063c-4621-a585-b65c80e931b5','62b18103-d68b-46eb-9bc0-6ee4507bd8bf','f22cd55f-b6e6-4d48-94b7-c6c3d54734ac','c18fc87f-cfc6-4704-89e2-8b5787c6ad12','e059a2ca-b3f6-4631-b019-893a137ae7df','f29eb047-8133-4e75-adac-35b31690a28b','2d409e4e-242d-495a-8196-240616580953','545b8531-be04-442e-a784-19bd19510671','f25e2d54-5090-4765-9c7d-44c7d4fdc93b','59a24140-fc56-48eb-b0d0-1bda55fd1988','834d2506-2417-40de-ab02-22026acfc31b','a470421d-b4d1-4f37-b4f4-41a11d6a4889','0ce1ff25-9394-4db8-bedb-02e5994f34a1','be9234d4-048d-4bfe-8f7f-848cce2cb668','1363ee78-be14-4c8a-8147-603550c53332','eb87b3e4-b10e-44d4-904d-6c42d38be446','c2e52f8e-8960-49f3-a2f9-32452fa5cfa3','096db5ba-6bc1-44a1-9604-8210c1d61c93','cecc8ab0-6a1e-44a9-bafc-8f9a2734ad89','3426e6c6-822c-4e15-8800-281370b85a13','267aacdb-4193-4f81-acfa-92400f5b05da','1b5a5ac5-e708-4650-bc9d-59fde3ec09f4','0e85e0d1-f04f-4cfa-ae19-fdd2d791573b','3f639785-a84c-4fd5-b5e8-b70c757c2e7f','bd90504d-430d-41b1-a0a3-572e9fcacb89','d24eac08-4162-403f-a57b-9d824dfd5f72','7a6d10f9-5cff-45fe-915d-1452872677bd','c1d5ec58-f5e4-4d80-b148-aa3ba429616b','5d8b7fe2-5aa0-4a82-9ac8-776eb268c642','892488ea-17a1-4f7a-8985-89abc48ad61b','5424b5f1-5e46-48d4-991a-867faa13bc4c','31690005-9ab8-4b2c-b36b-2f6ea4bb9ed0','095b13cf-c7c1-40f4-8db0-f4a2049cd6f9','f11e2cb4-8335-488a-a314-05c92ce57f97','0795b32c-7004-4e66-bff5-2ca4f0c9155b','dcd7fc70-c2a3-4099-9652-6ec6dc7a8acb','eec984a6-6b36-4e82-98e4-ddc8dfd53b55','6bf422cd-84f9-474a-a8e0-86804fa001f3','23a1bd33-df5c-4acb-ad2d-6e36d7872f96','ccf279bf-6b1b-420d-bd94-17a955d84e22','6d262775-2629-4e87-bd21-3608ca464e8c','1beabcd5-483e-4f09-8610-d4d4a19a52b5','a8c135dc-522a-48de-a16c-a6aeaf71c301','91453bb7-324b-4f9b-be69-6e97b188a1bd','9c974566-7f28-4eb7-82b6-1c9f5e4235ef','f8468c00-d33e-456e-bafa-df56a32a6f19','3d5bb633-abfb-487f-9461-0781e0f87176','b5b1483b-2e2c-41ab-a078-c2910e65bcf7','8f919b31-5c0b-48cc-a39f-c0fdb5ab26c2','5b42482d-51a4-4b9f-b95f-60872c157554','bab7336e-e0bc-4b01-a074-8cc24a87f92b','07766462-84df-4b19-9e33-826a1ebe808c','406a7d73-cc75-47fc-a4dc-904bc94768df','1e8b513e-2da7-4c24-8bc7-b6cd03e24379','e63642d4-343e-4329-b681-398e0eaf0e44','ba0cdd73-8d69-4a59-a0b9-a251f1afefc3','49ad8c58-708d-45fa-8f6e-d94bf822d718','a61b187e-bdc6-4012-b322-9fc4a2234480','8b27814d-6ad4-4aea-b607-a668ad7d773f','ae3ba6ec-4a0e-4db8-bb19-3f7d8f0012b4','94bb644e-e55b-49d9-8ea6-23f9f4efcb8e','77c68f30-eba0-4fff-8800-ae1d88ec1642','00bcb2be-b19a-40c9-af50-0a1d5211f315','9ed9d45d-8e46-41e6-a4a7-bb76ad6c5ebb','9fcfb0f2-f2c3-4a39-bf22-a8d0b85ca115','0432ae4d-0f5f-4852-912a-e22e71f64c9c','c7e2d1f7-2766-4fb8-a4af-03b1c8cc06d3','4ab08318-b449-4452-b138-48ed6723e3fe','559cee84-d829-4753-b591-8be5be597beb','7bb20072-a01a-4abc-80ee-55c579b87f9a','6eaac731-0970-49c6-b6fa-5dad2f977b66','d6090b9e-55e4-4313-8ae8-500497d8102b','94c853dc-367f-415d-8596-d42851646ee8','8c3cd7fb-c594-4b4f-82d5-558cbc42d99f','edbd3aa5-8725-45cf-950e-ee8fb14b9bf0','7c7fadb6-4d45-49bc-94c4-35cdd2ebeb5f','a6dd4c15-86e9-4253-8e93-022c21c20d3c','ea078cb0-7a06-4074-a4b5-479aa5f70c1a','773f27de-0c92-43ea-8555-08a02e1b0a06','1d2b35b2-e487-448d-9759-cb49b3e70b0c','9722d03c-069c-4d92-a4f6-a35c352c675b','bcc3dcda-9788-46c0-8b86-162a7a6c0e3b','0c4e4726-1d68-4f05-bc8c-c9bcad650e66','df3d2184-ccf9-4d21-9126-8b3a15d70e98','6bbaaff1-771d-4589-841c-ef44918179f0','3de7ace9-8af6-49d5-88bc-faa9dcad2c10','d87b90b3-5884-4f3b-8232-c7f2c3b0ba28','59f9e6c3-5e33-4ef2-a68b-40ef9789f7a9','43cb52be-afef-4c4c-8e7c-9e27e322d7cf','c65627ae-2909-4c78-86bd-c5e442c50396','d018ad00-5ede-416f-a83a-d0ba66e6f621','5d4b86e7-5b3f-4518-8477-f80e05bfcaf6','a022e363-d484-47ef-a573-0f5f94245720','43b8d071-f759-438d-9a59-ee4ea91e8ba8','24d5636e-1a29-4450-a527-7c9ba0ef26aa','b9bb0950-9820-4a74-9fed-89e8cf5ce032','ddf35e05-f2d3-4c55-bf14-eb9037e30918','8d9b90dd-1aaa-4b0b-a3fc-7321789ee263','79e500ea-faec-4cd3-88b6-1f0ddcdbe856','ee3af996-f2a8-4652-b166-acdd55842e00','dbf126eb-64c9-41b5-80d3-eef7f9db50d5','d5d3cd42-4b4f-45b8-b3b0-f1e436255e7e','ddee7eba-b733-4ba4-8482-8ddafdaa6669','f0dc9e14-f2a8-4747-9bd5-3d3a14b84be3','23a3d062-76ec-483f-9a14-810a66aeab4f','df5ed477-05d1-4520-96a1-9e97bf692ed6','c816ef74-6cc9-440f-829b-cbb0809a7149','23c3aa27-eaf9-4933-b1e4-5889627a750e','eada707b-2b60-4040-bfe3-15a9e863753d','a68e3cf2-1d08-4075-84a9-dc3ee1dd3560','27b59033-77c8-4623-b277-021db69e2c01','60d5d9ee-4cdf-4bbe-9357-0296c634f400','85f92eaf-e221-48e4-8118-6d8b8e114529','ae776e41-66ae-4eb4-b747-66849bd2ac36','aa0d2249-f6b3-48e8-94ac-ff42bb3998b7','5c749ae0-899a-429f-8d75-9098ba182819','82acf532-76b0-41ee-a4ef-7da40ba3bf1c','e865d960-64f2-4a0f-85f3-c57f02174323','381a382e-0c7a-44a0-a0a9-c8c68ffa78df','3640145e-57b6-4d88-8ed6-49c965857bc2','71e93cca-790a-4ac1-80e5-216ea35fe0d9','450e83d3-2c07-459a-adb0-1555f0de2721','009ac0c2-86e2-4fd7-9f3c-bf4b4351b8a7','bec49ff8-b980-4805-83fa-49d37634d86a','f84960e5-0cab-4227-a8da-5ec880659500','90135805-e29f-4796-b0a6-9afbcdd0b6c9','e8a5c227-babe-4317-beae-510af734303f','c8dec57f-cecc-46df-ac8f-10a728b4a949','76b51c16-9422-4b4c-b271-0f9dd79e212d','4b3af504-ecc0-490d-a1c3-780c91c87636','ed046a8f-95fe-4c5e-9099-743d2dbf43ee','5b1f0089-dd41-4fad-8d27-61ba9d334ae9','1446d753-3686-47a1-b6c2-c4dff7a7d388','c21f88e9-2171-4a1e-aa33-c159041ac133','dc1f39de-fb5d-4f78-84aa-c58cde8c2fbb','1ad53963-9aa6-4a14-b4cd-7bcffb61c1cc','cad8e784-e458-40ac-83f2-4b8535f8e9bd','738cbb55-908b-4edc-b7ed-50a7747b434a','710d23ef-e540-49b1-854b-ec99aff3e39f','d460f785-99ad-410c-bf2a-6ef9ebd049e7','6c27ee24-c63a-4572-9b38-cf1a06162160','655b4537-e86c-4054-a080-1f998f7c9fd8','c83dc60d-a605-4b97-990b-7b45c1f310d6','a2319d95-2de7-4205-8bd7-013b5e18dd03','2f3ef123-b1f2-4dd7-b26a-f167867cc5ff','affe6e53-f824-4703-b515-017d6afd0c26','002e44ad-8c85-4945-81fb-2422bdbb26d9','636ece47-ed5d-485d-a3d7-54d66196f4e2','e1a0ba21-6bbd-48b0-a942-b8a0bca86af2','bae897f1-95ee-47cc-9f21-f4a9d717743e','1d34256d-b0d0-49c4-bf4c-1ddea195dab3','0be41c6c-7c40-43c5-8876-dc448f76d185','25ef2894-0154-4a46-acc9-6dd9825266dd','d18d7927-61e7-4312-9b9e-215b6d6f7d4b','fb309878-0435-4db1-92ba-b6a22129eda8','b58fb0eb-4afb-4ad7-98e2-ca871bc2a6b5','1639e90a-fa13-4384-96e2-e97f435a6ad0','5e7d11c6-5e4b-4e07-bde5-66bf56145e2d','7cd0ea68-bd96-4cfa-9b7c-1f854fdf7449','81e160ba-5f88-4650-8d05-2a3cc40b8df9','46358842-300e-4d17-a8d7-24b096ccad34','ba3d0f79-7ea3-49c7-bf7e-51f37083a7cb','054b1b28-52c3-4ed3-a4ce-25b55390baf5','d0953574-22c6-49a0-9ac1-d41143a37b88','bcab80d7-1c5f-4809-af78-681487caa310','9d191d52-2cd4-46ad-85b0-4dc2100d146e','d15b80be-09a8-427b-a846-ec350530ff11','c56e44e6-673d-4d74-85f9-36b734f19b7c','734268b7-e21d-43cb-8050-b3219de564d5','05c6b2e2-0d65-4b68-ba7e-d8c5aa34e4e9','79242be1-5ed0-4517-8f87-3e0273f1b0b5','d9d04f0a-0b78-4de7-91c0-1487b8da89fe','913f004a-65fb-40a3-8488-00e07305d253','b58644cd-8d9a-4c1f-86d7-4662fb6474fd','332ff986-82f1-44d1-ae8e-52cd59c0b068','8cc8173b-b928-4e83-830f-ac8224b95919','65ea4381-e51b-4bf1-bef7-872700144802','443bf7e9-f9b1-450f-9d2e-05a2f55e25a5','ae2ec427-3f6d-46a5-a448-e81009f8918d','a8d20fe6-0b05-4ea6-8d56-39628b2cc258','7f7de9b6-647e-41b5-b2d1-b31af66db556','d78d4e91-fce4-4dbe-aa89-1aa1903bdb20','955c42dc-7632-4b96-ac0c-85df67d82b79','24646e58-fd29-46b8-aa83-4cace17f66d6','637c063a-9f6e-42a7-b53c-713b1c33dae6','63cdd2ea-88c6-40c6-9fc3-d5cc3324c979','e39d5662-8616-4f5b-9ed2-a4d1cae9d668','008763a5-706b-4fe5-98d5-3f0a77976c9c','e8aeefaa-c653-4aba-9ba0-c799707df5b4','a5ca1d88-8ef3-4de4-9d77-9245f08f049e','a1d7e655-1312-452d-91fe-b1733d4c4c63','eac4abf1-dfc9-4368-bc1c-c6c1a923cae3','423bcfec-9839-439c-aa84-205904c46ae7','f2dde3b2-83d7-4694-b5de-94646012ef78','f278ea96-cca5-44f0-b011-0813a180c773','a72802a4-9c77-40c0-9569-502f88d6525a','085852cf-33fc-4805-8b6a-cf90829d3d18','db6be3ac-9e0a-4188-8a56-ddcc1f12c089','6e574f36-8ba7-4201-8ae3-e55311ecb2c6','41269b9b-618f-48bc-bb68-83bcbd32866b','f039eff1-0a94-4685-9d52-088c085bd420','8f5229e1-3a44-4f52-b36d-f8d42a5722d3','6cb146ad-5dfc-481e-a67e-6c8b58e4f4bf','3698c709-73ff-4dbe-805f-83a1f2f54682','55336fd7-1a0a-4faa-a1b2-13dde1827f74','e678ab82-b042-4972-b993-f3eb1013e59d','b977288b-f764-4489-b187-062fe8f6b772','75842a4a-ea62-4478-8621-0267c8ae5831','dbfcede1-e306-4896-bee7-d251d5c9b916','11fc2e08-bd3d-4af2-8925-46a44449f130','e3cb540c-118c-410a-9eae-52c5ac0033c0','245adabd-1e9b-4808-b157-ec4dcf3083be','8fefa7c0-b4f5-414f-a9be-842f7c608bca','4bfc4d9c-46dd-4597-8906-bfe288f76730','a5e7227b-d3f9-4166-aa56-9fcf100bfedc','51390f33-7b45-4e8c-86ba-d808db884cc3','e545c139-8381-48b9-85ed-77ecc8a7cebb','7c46fe10-96fc-470a-9d55-e1d22ce5e97e','acb3bf81-47f6-448d-9920-287b5f25168d','a6f424ab-5192-4b7a-af94-f648e23c85ce','a1505565-a69a-4845-9670-080a65ea0ff8','c956b902-537e-4cfa-ba00-46aa23c6cee6','a87943e8-0c0d-4c9c-b5d2-e30abaa53ed1','8458dc3d-588c-4455-8ecf-38adf32eda0c','816262c7-2f40-4ba3-9c4e-d7fa056b3048','26b773bb-ddb6-49c0-a6a6-dca25a84f423','9f7d5adc-1488-4ba6-bbf7-17d4e5daa8bb','56252626-7bf7-4e92-a462-078e41c22a46','be12ac92-7b14-4b3c-bab3-79821e322112','81fcf438-1a21-4ae6-aaea-faf4a9d0cc1c','4ebaa966-997f-401c-b0b4-a2ca720e498c','83dc7463-720d-4314-a3d3-59d3c44e7ee7','9bb81d10-1e39-4eb4-9b26-c658e42a4100','5acc3ae1-c38c-49aa-9ad8-bff2f9ef3c6f','5b82734b-f799-4e05-8b63-9327e6a526ba','30844610-bb6a-4c0a-8234-a64aa833a8bd','b131f7d9-7fa9-4f70-aeb5-2403f5252e9f','88084f0a-593a-4e0a-a49a-3a62d9dbdaa2','727c492d-52d7-47e8-820d-1a22a5ac1628','9f521301-6caf-4ba9-b932-aae842e4e75c','8e54dfa3-5324-49f5-85b8-f32b45de4ac0','da7cc8bf-fcb0-45e9-882d-def5c5cf3617','dd7fb067-adb5-42ad-964e-e1d23e5bd999','da4a05be-91e0-4427-97f6-e925e1403f66','12049dc9-657c-4309-9039-f526d3f85d93','59f9b16e-5519-4b18-93cc-d21d344e5f30','bddf7c49-303c-441f-b5d4-6119eaa2a304','dae46c22-4eaa-45f2-81d0-b657f5edb1d3','3c3e00b0-4640-4595-a8be-6f35d7a710a8','d0939f02-b3fc-487a-bbb4-c8e893019fa3','59c33f1c-af97-4d37-b864-99245018d978','b8ced120-54e6-400d-803f-7c5ac746bcbd','39334aad-937c-4abc-a300-d90c113c6d6d','d1b1b9af-6ea6-4df4-9bdf-2bfcef297c28','e7f8088d-04c5-4176-a2bc-783c2205ed55','3ea06c48-09e9-4e15-9cb3-3faaacea24d1','83f47e19-5c79-43fc-8051-f0cf528b0392','52eb2c07-5b98-410f-a8c2-26032667580b','e4a24ee3-e617-4091-9f74-92195257a1fc','22c64c3d-9449-4b99-875b-ff581a8686a7','bdd51fc8-987b-4c13-ab39-cdd27482743e','d18df271-19e5-4e83-87c6-4e03f96fff3b','29bfb0da-494e-44b4-8378-1219f357a776','805d3947-572c-4a96-8278-3d4d2455b1bb','65ce7db8-a413-41ae-9951-b6b9daab5cae','8fa9dae1-e82b-4bd7-aafb-a76c7e304ec7','694d6348-a523-490b-90e5-0e3f748d910f','eecf5daf-0bae-48f9-855b-b07f65797b01','57c8a049-4352-4fa1-9dc4-d66d391afd9e','319b2a77-76d9-42f6-b53f-41c44291a675','cdd9249d-dd0e-43b3-b747-2abaa04a4ea3','f54bf985-9ac3-4037-b641-61d8f21f5c2a','defe5d02-36c4-4bdf-b67e-a2cbff9ed4f1','7a40f970-d3b5-4615-8ec3-64006569c447','cc14e0fe-4b45-477a-a82a-61bcde76758a','d8941e87-b367-4415-8e38-e89a2ea3618b','352ee4ef-522d-4b89-b8e1-a8d223e08ef3','99867b7c-3dd9-4623-b091-1e5bfcdf0668','7d2e69de-17ad-4453-a26f-a384057ea511','25829eb8-582d-408c-b2b4-729441466676','c74a75a2-822a-4d0b-b06e-e9556abf682d','c3383be7-f5ea-497b-b84a-d7f939029e00','5029c326-c91e-4df4-af62-b7b487e38f3a','acb97773-4482-4615-a337-d8612ac82985','8985e81f-463a-4fe0-a666-8f90c0a5d2c1','f085f57a-25f5-4735-bf4b-a6a8885417e9','795540a5-e0c4-4bcb-a586-ba7f1689890a','d9388e50-f288-4e35-9448-01e5a084eee6','32a73879-6195-4a8e-9a0f-ea6dbe5be471','0c1c302b-b2a3-4daf-af4f-cad1f88aac14','a35e8f68-efd1-41ed-bec0-ae9b24d7faf2','eec84476-15a4-4c8f-a2f9-c14f969765f4','79a21856-23b0-41fc-82de-dc5d1a99a69b','6cec7c24-50b4-45e3-9783-40cef23098d3','79107c6c-0156-4150-802e-a1030ea48f55','928eeea3-d78d-4a73-85b3-9e54f87b26a9','0e4006e6-cf51-4c0f-932f-8ec1e85dc8a2','fb806d85-e812-44ff-bca1-13f156ce0017','62220644-cef0-44b8-a860-9f818c650a61','adfcf317-8ca2-403d-a2aa-136556a06ae3','be408c54-2114-4291-8222-9aa20482dbb0','8571a4b7-dbfa-4098-afd4-544649d4bb19','9baefa26-3d65-4c70-82d5-5f1b9e6c1761','0af16659-8c60-4817-8d88-d91a7a51af3a','87e812c9-db45-4a31-8fcf-7ac8b2adfd6f','7567c4d9-3f41-4cf9-95f2-0e37bb80c36d','fc8ee809-24a1-4518-af99-a12eddd00f02','03bad5f5-9a67-4b09-9c1e-abf7d6ba0958','83f6ed59-1289-4fee-983c-7920522e966d','89c5a7c4-b027-48fa-8f56-406fb4f8c7a9','898afc4e-e4df-410f-8381-a89b469c8757','82661df9-ed57-4188-aeb9-c6e58aee3c8b','b948e7ae-f945-4fd2-9884-393f6ec62134','03007c10-bc29-4e2e-943f-316065c8e4a2','b6a05235-6022-4d22-b724-372ab3286881','d78ca79c-fe32-4664-a3ff-8d62b085887d','1825163b-2f8b-4841-b6ce-26ac3e41d96f','7d5fa5a7-f4dd-4d9e-bd2f-b15de09667f6','9690e668-172f-48b4-9527-2e6823f3fa82','ce349f5d-ec34-4156-aa74-9b2a42481e8c','01783611-ab4e-4634-bf9b-d635fd7bcdaf','fcd4bb30-ca28-4a49-922a-f8174011d9b0','63a1a333-eda8-4d23-931a-90de2385f0a5','c37be56a-860f-4de9-9d05-7941c2b84b0d','45a292d4-281e-42e0-a50c-0cbda7dd4377','f71f13a8-da87-449f-a056-9a2a3237f3c3','70943b36-56f0-4155-b066-46b8ae1cc53d','d70537b7-bb1e-46e8-9026-ae8a8513d2f7','5f91c645-1bcd-4bfa-b9c5-8807a7081b30','f36753d5-f943-49c9-a601-664955ae2511','339f000f-8bec-42a1-b8e0-30888be13754','6c1ceffb-8dfc-4d70-b1e1-28b2b3198b5a','2612aaba-eaaf-4a13-8b01-edd57674edd0','38535784-df4e-4a7a-af79-bfa85929ebeb','da6729f5-0a10-45de-80ac-ae232795efa3','491ab495-fb63-4b28-9213-d5748389e408','de5caf16-ac4c-4267-a023-6585a24ea5e6','61985538-9dea-43d6-b3ff-3ccce3a2b76e','a5295552-abd7-4e15-a567-152c679d8fbd','ed6208bd-f33c-434d-825f-2df3e56fbd5e','97a9e35a-038c-4079-8a66-7f32b1947409','40e11a3c-e894-4fd6-a956-075dc0353ef8','f088df60-1f34-4abf-82f7-2b8bbb3d936f','b304e696-a2ed-4b63-a5f4-2b9a5e8d72a0','9311df22-a32c-441e-b163-5b4c89d93928','b535aceb-2016-4ab7-8150-11d1971976c2','8d8d6973-355f-43e2-93eb-48a4f4d6d3b4','b1e16be5-fb97-49be-a048-f5c9f3c0bebb','94b89f70-0089-43e7-b942-03944791b245','2140e58b-6b32-4e93-8a01-2ae10fc82fa7','bf644eb6-c992-4cd4-a1ad-a3ba698daae7','4f7478d0-1f81-4d90-a644-0f952613d285','61aa8f52-848f-4d61-beb7-ef45ff8f16fa','f3851ec9-8848-4437-8a09-dc8bc362c774','9f218308-85fa-4b50-8921-460b4ee13720','4ae692e6-685b-4ff4-961b-53a4d144622e','1d1c28b5-242c-47b4-9a35-0d124ad289b5','1791af50-fd73-4b94-a705-72277a6e4dbb','9b6ae3d9-e240-478a-8b84-8e9048c2b3c3','809f415e-9791-4ea4-a1da-c6f6ded07bb8','90efa9f2-f841-4043-a4ee-0cebc84e8812','208306f3-d67b-4e25-8e98-64a1d87a7dd1','3bc54ef4-0b06-4fbc-b879-2dd50c6cf401','c4454fce-439a-4d68-bece-bf5c2ff34279','923feb96-a2e2-485b-9524-89140e1007ed','a47857d0-6aeb-4962-a9f7-6940a02e8ded','83a29b24-0ac4-437d-a4c2-a99789335cee','5bd49592-6228-47ca-82f6-0f9a166fdae0','3f8415a3-8da4-404d-a78c-c67eab734dba','cb5de22e-d272-4b91-98e4-7ece4783144e','62a7c108-7c48-4766-87ae-f297546b81cd','38f4b873-8cfe-4887-a50f-09eb231e70ba','9c4ec4e1-a6b6-435e-bcb7-32a8142b2f08','23dce82d-4a55-42ed-ad74-e65749143d13','84dc9cde-e0df-41af-a484-91b985c4b0e1','fc37be05-1572-43bf-85e4-5244f038edc3','b81a70ea-9ca2-4059-8682-51f6310767bf','bcf26268-e245-47ea-a75e-8c696424920e','30571e5f-6a23-478b-907d-41f0a37d9095','d2336817-8b6e-473e-a07a-7f67708531f5','d29dec84-077f-4506-947a-8d1190e0dd35','99c2a411-2983-4001-a341-a692aa82bfe8','f0205cf3-eb28-4f83-9121-8af398277b1a','f1a2e8c0-39de-4444-8b12-848a4f43e3f5','ece5c6fa-0d2b-48b8-8eaf-b6b337ba9419','e4479c58-3586-4c5c-9180-b7281c716a59','29812681-0b01-403c-85a3-cfe731f38b8c','fec89714-d5b5-46af-822d-85f01f1d52cd','cb6520f0-57b7-407c-85a5-d69f960af688','08d2b437-1243-4522-84fe-913ba6bfbd31','0fb6b809-e260-49d6-bc73-8add4ae1c029','84c5cb0d-a46a-4158-bb39-a6305ede2d7e','7114854f-b98d-4455-8fae-2998a1a1794b','acd618cd-f1a7-49db-a251-b5b6fa9a628d','be97ba0f-ceb1-4ffc-b352-402cc0b0a03b','e048b0ee-4622-42aa-8242-709d01dc0dfd','5f5d9629-fffd-48cc-93ba-f868e4f37090','547b7a12-618e-45a8-9a2b-c76ac9c5ba18','d68e4e04-ca54-45f5-bf8d-024ac2dd8d6e','0ede7b3e-df19-450d-933d-5b808ddf9237','a58e526f-74de-43a6-96bf-6666a0ddb26e','40e2b64c-1b66-4852-aa6e-fbfd4801df13','2fe60ca2-1309-4a4e-b7a6-f3e305d503e0','8a70e571-e514-428c-97dc-3cfc8d06462a','1ccc83d9-5172-4286-b0a5-0f56c8f69b74','75997f0b-9e6e-43be-8cf2-4c4e93621693','2877bb90-6c79-4a7b-9e91-dbcf2878a9bc','d6e2e8da-ad6e-4df5-a53f-3c97573f6181','d4f6730f-d70f-4037-af3e-a5ba6b211205','7da4d2e7-6a9f-477e-916c-40f9562761ed','681d8f97-6f01-4fc2-a200-967a73fb270a','28c8e89a-70e0-48d8-9b3d-9875f9e0415c','c1c96a3b-ab7f-4190-8bdc-70944e646411','a17002fc-cc38-49e6-9752-bfae15e83505','569aa035-4ec6-41c9-ba2f-a71c1402c4d1','3a6cae0b-bfe1-4009-b046-ec572981cbe5','48758e5e-4cf9-4ec7-9ce0-2efd008702af','cd96c8a9-302c-4c7b-ba72-fd70198e9ebd','18ac4d96-adcf-49b4-9c88-1e468a2e97c4','35a39600-51ed-4772-bec0-a83c98e6b248','237f83e3-6ea3-44f0-bd50-00a8e092f3c1','ab374de1-454e-408a-a769-0ec691f3e827','d9936185-4651-4937-b0e4-912c72127414','4fef5522-1852-491c-b56b-1753a22408b6','114be60b-5f7c-48d4-96fa-98cf21c587f1','5289112f-4796-4c7b-893f-da047f7b8e9a','35dfbc81-1311-4883-b686-b8b6aa473456','b10e9a3e-7458-4356-8045-613180ddbce1','c957e88b-5398-4eb8-b778-72da14456a39','e6c1249d-3a55-4e12-8813-ed4d56d101d6','50fcaa3c-58d5-4f6f-a502-8f3d215d6f62','cfe04beb-c78b-429d-b6cb-890838934170','7a4f6d3d-3087-470d-a538-014dbc493aa5','cfa07369-acab-40ef-b904-0a9f03d41122','d2fabf52-5e09-43d9-ad5d-62079410b135','317ded16-13aa-4cb8-9d05-848fb35325e3','5fda8a55-8614-4db1-bd37-2ee1c08ba95f','06dea062-43c2-486c-9b36-76267cf9f8a2','8d044ec7-3b7b-4cf8-8d43-ba82b6c957b8','7fe5b724-94be-410e-8616-a77030cef0c2','0f1541e3-6ba1-42cb-8f1e-ce523383351f','4def5784-146f-4bcd-9f32-ae5db4914810','ae558b23-6584-453c-984d-1ac5f03c953b','83bfa7ba-6c3b-41b5-9688-fccf7522e036','59d2da11-4e26-4ad1-bec7-6ae3dd31548b','637349cb-b19a-416a-9f29-c5a02c94af5c','c585f9ba-4e64-477d-be54-bc6ff7ee4213','6ec1eb69-0c38-4556-a306-6c09385ce375','38406455-27cf-4736-aa38-7a5117f1bbf3','827348d6-a959-4803-af30-2788cc1a049b','5c0ac611-5aa8-49d9-9f96-504d115e3778','00359e90-e85a-4cf0-a7ff-e2e4ecbe4172','9d992a4a-b329-4c07-ac51-9f629ceb7c8c','80d69300-8e52-45c3-b74a-44878ac671ac','3153a8fd-f80a-4e3a-87ae-285991e15734','7346d84f-227a-481f-a600-cd2fd8c2ef1f','3ee0249d-97f5-4dbf-8f0a-eceba42a154c','8fbe0660-8a3a-4da2-9b44-387b91c96d0b','ef4b5a09-3024-464a-b895-c30828ba53f2','328de418-526f-4015-b2be-81fbc4057595','ec1f99df-24f3-4e55-bdf9-e4e85cd7bc39','5d68634d-6232-4d0c-b7c9-2111cde7a90c','8e1c70b6-cd89-4bc8-8ea5-37e0767a9625','1e59b9d2-1f71-458d-8adc-195dec8886de','0fb4f5de-ed22-492e-b59b-a97ea6c76554','b09f47c1-9ed4-4222-92bd-c627db46fefc','f8974c88-09af-418f-a007-004753730d8c','4323ca91-6866-4711-8e94-7a23769ed084','e6bc56ed-3287-408f-aa19-7dfd77caa23a','b70b0097-04fc-450e-981c-ffe727edf665','96f95b42-bf44-4e30-99b8-a290fa3e6596','4dddbec8-26fd-4845-a8cd-b28665a457c7','b6e2b324-8189-4e7e-a98c-2032be4cdf27','5c7f6c48-a6e1-4c18-9373-b9935d889aad','131a8881-c91d-43ec-aac1-ce8116b40874','41066a11-5712-4bd7-8265-d409d1cddfe8','ac69c92b-abc2-43e4-868c-d2d2828c313c','e3b64adc-25d5-4df6-91b8-1b0f372650e7','f07f54a4-724b-4a99-8262-2cc86944084d','6862e605-e26e-4b7d-a0e8-0f82d3672cb6','b3552f1d-4599-4735-846e-cafe49717d5b','7e97ac4f-58af-4ef9-8374-670e1fa9e76c','9c8af566-113d-4e64-9c9c-5661f6975e95','fb49df21-35bd-485e-ae77-9e1eaad54d96','84a26f74-4168-4abe-bf3b-6e21978d9415','eda9f79e-84f3-4bd4-a58d-333876346d63','69e5ddf2-1b74-45fd-92eb-947938bece25','7b695739-7a0a-40bc-a39b-8049b4e78828','432bba9d-ba23-4014-936c-24759aceeee7','52c50e47-d9ca-4de3-a222-16217de9b877','c93b15f6-3b2d-43c1-8588-691f996ad722','613bc8a2-d90f-4fd4-a759-65375f956e94','c10f4956-70aa-499c-be4e-8e128d9544a7','d6f0199e-6783-499d-8ca9-1b8b5f870564','013fd465-71bc-4131-8b57-bf9dfe52f70c','1aa552c8-4d24-4f72-87f9-3bd381ad15d6','0226729c-b70c-4fb2-a848-af15dc4e2205','b701f918-ce50-4e17-a501-983e689f87dc','df168f0d-f40a-4323-a906-a4890b87e13b','0577853f-512b-4b73-b18e-ff82e08fc749','46282722-90d3-44b7-9c82-b5dbf5958b21','5cb2caf1-13e7-4db8-b8a2-1dc6e65589da','2e4ec7ea-73f5-4261-b4c7-2ceda5c0a5d4','4be71a33-1eb5-4867-a5d2-f90f34ad7790','3a29a010-5f7d-4933-ae07-7993a3e5b0b9','844e0a8f-9297-4a5d-9d66-9686783a0c77','b2adcdf9-1aaf-4df4-9511-92e5a4f7c60e','aaad0d64-3a94-42ba-a8ad-b32a01058414','84038f59-ae77-469b-b0a1-3a84e34a8780','f2264056-6416-4235-9426-2137299cf029','abfe359d-d2ea-48e2-a7b6-085f21f7d70d','26e58fe8-6a29-45c6-9f4f-04247eb4998b','b4b7b64a-638b-4bd8-8316-4bc9dd91a20d','05460559-5ea5-45e5-82c5-874adb8b6bd9','9639bc12-3cd0-4fcc-bbca-3603d5775342','1b2b2a52-bd42-40d5-a4f3-76ff24297947','186030cc-dc87-47b0-94d4-110f188aa2ce','ceb86c11-a824-400c-85e6-bfd76ee47857','8062abad-34e0-4a12-8bc2-2cd3ac21ac3c','909fc645-498c-4f2f-97ce-75fa99a21327','d8d6d0bc-f3f4-44dc-b006-b0297a2e2856','50dee087-aae6-474c-b66f-047f62d2bba5','7fb75f0e-b506-4af2-8954-bd93cc50a9b6','ccaa7373-3cae-415e-a04d-26bee4299977','24d80be0-ec07-47c8-9ee2-7c4bbe34cd51','11c92d04-6cd2-4332-97c7-8f451aadf989','baf69e37-aa58-4962-a161-e5719f6d1528','d93490a4-8a6e-4bcf-9c89-35efb97ca688','343bedc9-4d48-440a-b563-aefb706a4a5e','974b8527-72d3-4891-bbf8-655c77bc7a4c','1690b6ef-633f-4cb5-8368-23af6c6b79ee','efd240dd-cd71-49f0-817e-ad9bb5da0d7c','2f93b24d-733e-4557-8b1d-a6b8ba89cd8e','8f75c703-13cf-4e5c-85e9-99b22be38711','cc36a110-1ac5-4b42-9072-5b4f513d915e','ff64b55e-2c98-447d-a66b-9307ca9a0a98','d1ae685b-e522-44ba-974e-f9d0d394ed40','207a3285-2d3f-4ac3-8da9-25246e790a05','c27b8917-cd9f-4d01-886a-fa85c86a8bdc','daf7254e-864b-4f8d-96d7-741bc401293e','e8304d6a-91a4-43f7-a8a5-1df383b2ad2d','c5b5fdee-a1f8-413c-a1b9-27bde17d0ef1','e2ff3433-f83a-4c68-8e61-cb74ce879063','0c5d689f-bad0-4194-9dba-173269fa45de','e36a64dc-f86d-4282-bd32-a046f10785db','e1b42db3-ebfc-4afc-8b7d-edede6a418d9','a62c5bb5-2b43-4bb8-89e7-7c820dcdf26e','f18efac4-08b5-4117-8e14-7788965a1558','631826ec-4a77-4430-84d2-49cc88d8d84a','4dffdbec-027b-44b7-9ea8-2800fd5d83a6','00fcafa8-e89e-4b89-9179-374a5ced8c52','4c6543ca-37cf-4932-a814-e7298c75d0f8','954c5468-1894-4e95-906f-41d685490bb0','83926622-9f0f-4a16-9af5-87c35087363f','42d18a4a-03db-4200-b6a2-2ad67ad400d4','722935cf-03af-4aaa-b239-77c777d9baa6','b1563189-68fa-4e7b-8184-678d494a7069','e7f46f4f-9eeb-4270-8085-6c08afd0097c','38b04078-1bf8-47ba-8b97-c2e2c37b10e2','7656990d-a97f-4001-b31b-782e4d1f67f7','ab9e3e1f-159b-4433-9ae5-340032227d6e','1658fd4b-2e4e-43ac-a9c4-dbe44c192583','594899a3-ba4c-41d3-b269-cc2bd5dfbc1f'}}),'92362',struct('BlockId','5f2025b8-49c9-4174-a50f-9954f6fd5e3f','SignalIds',{{'62732959-251f-48bc-bb75-6563641d8800'}}),'92364',struct('BlockId','c5b5a8a9-c0ca-448c-8db6-cd3c9b66be1d','SignalIds',{{'6344fcee-de29-4e13-9955-19d1b344181b'}}),'92365',struct('BlockId','3ece8d90-f93a-46f0-9ab2-53960762ed99','SignalIds',{{'cfb6b582-641a-4870-88e5-47bb370f67ba'}}),'92370',struct('BlockId','1d9a14ab-e7c8-4f8e-b2bf-038c92befc3d','SignalIds',{{'b73568e7-b091-4dc3-8ca8-153143d1aab5'}}),'92371',struct('BlockId','7fa2fef5-94db-4989-85dd-77beb36f0834','SignalIds',{{'1dfec191-1e97-447c-b39d-1186a18f1d1e'}}),'92380',struct('BlockId','e7881de2-179c-41cf-9bdb-b87de17e3ea7','SignalIds',{{'d99500de-b16d-4559-bd0e-e6dac15a0288'}}),'92381',struct('BlockId','8780eea0-5b4b-4d3e-83b3-1728cc0b02e5','SignalIds',{{'20014170-9a8b-46d7-8859-1368f7d75241'}}),'92382',struct('BlockId','29917c35-f334-4b7e-af81-65afbf6f4cf5','SignalIds',{{'984ba9ee-211e-4012-8798-bcbe500a525d'}}),'92418',struct('BlockId','c5a7be29-3173-4b9a-a890-b4cee331cb8b','SignalIds',{{'79a90cdf-8a9b-4ccd-8944-69c4469088c1','35cd3c97-8160-4258-a864-27af0ad45a59','a068c4ce-1004-4dff-b2ee-cba0a0b81dfe','05630d0b-4185-49b8-8feb-e160bf4c7342','87327782-42c8-4aa9-829d-57e10c6a236a','32ec414f-0201-452a-a464-db511b140477','a447bd14-b398-4e67-a61e-10660811da2c','bec63126-1009-4953-9712-db8f6ef516ed','b2eff86a-b6d9-46cc-97fb-d1becbbdd2bf','de8cb12d-21ee-4317-92df-23379c880453','5f05ca3a-8a5e-4853-a5b7-8c6c0dcf0e8a'}}),'92419',struct('BlockId','793c2d2a-ebd7-4dfb-b311-846f772c752c','SignalIds',{{'c2b3d6ee-be4b-4de3-95b2-89c4c1a90859','2f308f5b-558b-42d2-ab39-a19d3bc85296','12894442-8f81-49fb-bc96-47a5bf1bca4b'}}),'92905',struct('BlockId','c130785f-a926-4d18-80be-4f90a56fc66a','SignalIds',{{'eccbb9d3-c00a-4fed-9913-c35dfd825c91','c1e83077-f3f7-43b9-b95e-2f4abc61ed1f','b3378ad1-fa9d-4543-8cd3-a0383f142dc5','fa304a37-e84e-4267-8828-303f093fe0c7','3e860a56-b4be-44fc-83d9-afae1ad41a3e','c999cc34-3a38-46c4-8a1c-1fefdab530c3','fc5850c5-7bcd-4c27-8c6a-9a1a118edd15','71bedb22-8fce-41d1-b1d8-8abf9395d0fd','fcd7fb69-afec-4b69-b843-6566c7a71cf3','2f9a360a-3789-4020-a595-682571a650fc','7d4b0e51-2c7f-4ae3-b318-9737498e94cb','fc0bc73a-b230-4af1-a180-3ede73bf37d6','766856df-e6aa-4404-a2f9-666f11b78eb0','ab8c368d-5e20-4365-a424-76159427f1c0','cd802434-50ca-463f-b66f-d14e79cb60c4','efac5cdc-3a28-4136-adbd-30ddc781af6d','db1258f2-8f31-40f7-8b6e-1a61acd62137','765381b0-de7e-4511-8d11-c54a539c85ce','4e1fdffe-5de9-49fb-9c6b-b6115907f89a','d47039dc-7492-42a7-b7c6-a1ab58c33c7e','d4300b37-a6c6-4c57-a896-906157398140','331d091c-d097-400c-846b-e57d9b47c756','23db7ee8-2e7a-4648-ad47-b037c2972cef','7a92bfbd-8432-4cf3-bba9-5102f8da93a3','d6225bbb-9586-45b7-8ccb-407014cc48c5','23441fad-9abc-4183-87d7-b259083607ca','0dde033e-7c55-4e81-bed4-f372f31ef215','19299d9d-d888-43bb-8f47-8e7058fcb5c7','224da2ed-8488-4958-b851-20093da22004','7efba0e1-16bf-4181-8536-a48b5cd2d0a7','e73f4837-c9b1-4144-bea8-1520a76a6288','39f8688a-7822-41f5-ad84-d137df05f1ce','13253221-23c6-4520-91d4-b12ce5c98f82','2b2864b7-66bd-4bf9-81c4-a366357cca21','8c2ff0d7-259e-4a1d-bbdc-07d0c2fd0dce','9c98bbee-a96a-42fd-9207-e63e410c9150','ff62db54-7a7b-4950-95f1-e767ae3f0f49','aabaefa4-1632-40cc-9882-d40a0daaa608','5c5c25ae-9e86-4fcc-9c48-44bf11f46d67','75186855-9909-40bd-9e53-cd5155d778a7','b2114956-6d65-4bbb-9e37-67f3500147fe','09c2ba44-b82c-4619-9656-42a1607dfe92','af2f1598-0ea3-4de1-b7e3-52d79c962171','fd707be4-0fa6-4ae2-9f60-4370b6144153','4567b165-8011-4f30-8170-b653fb7ca9ca','ce1b30b2-f922-41e5-b8b4-db9281ad7f48','981d4ca1-9a18-479a-8eb7-d9972585790d','2c9ecb52-7d2d-4aeb-9d3e-a4c1e8b56aa3','95828839-e7d4-4a62-bb80-e66eb611e1d8','a184c7dc-5258-41a4-8c4a-c1be98591e3f','35ccfa30-c7db-4b04-8d9e-77ed7147eedc','eabdcf25-6724-49c7-8252-2b7db0dc0620','9c5887e0-8426-451e-b3ad-01e654ac3baf','1ae96621-426b-45df-b021-87aa2e52cd1d','89e9c9d5-36d4-435c-8975-5c50695f6420','c37a17f2-821b-4110-be36-51aac86393f8','7bc58ec0-bb40-4800-a223-2e444648b98e','e633a30d-f132-4524-b75e-0d9f6e9215c2','90ddf5d2-13e1-4ad1-961a-537e55784248','7d166e16-84ea-4099-8464-ce279385cc24','198a9685-b37d-47d1-909d-4bdbb172482f','2d281c1c-a91d-4a00-a1cf-9fb8696d6c2d','7872f9f1-7e80-4cb5-8ed7-ff8be80c0e6d','9ba31d8f-2dc0-4834-a390-6e97d705a4b7','107d086c-475e-4b0b-a20b-5263a4427ef4','c3d66b39-b3fa-4845-b3f3-5e96d6860841','49e18595-2bd6-4e15-bc14-e9bb0458c226','2f88091c-fe89-4fe7-a6b0-adb380293617','bfe86deb-ef77-4a46-bc27-242d234016ae','72347ea7-d7cb-4ce7-afa8-b3b4972bf273','185e8e44-603f-44a3-b375-4ee1d80c6d3c','e6479db4-b6ff-4f92-bfaf-5af0158b2bb2','4e72e28c-3ac1-4177-98cf-6ac5a77a5b5e','d3e5cb8f-1aee-4ee7-ab68-88242de410af','d6ccaa71-6906-42ef-b48f-158ba10375bc','fd28349d-425f-4f21-84e4-1e9d232cfd82','a8d07bdc-79da-48dd-95f5-7ed7f0ef04ca','55b165cd-91b4-4efe-b4ec-5ce94f7b842b','65d838a5-3c8a-49f8-8107-95e629dfb205','36d6d967-3880-4484-8ff4-a86fe1881e48','f6c72526-ce4d-495b-be35-b87b229b2ba2','eec45291-cc04-4e1c-a4ab-647c5bfd71c1','4b49273e-9e1b-4ae5-ba38-9efe2ac32757','a557b5bc-8dce-4849-bdb6-0dfbd7ad1634','f827e4a0-73ed-4c19-a1ff-1dadc01fa3c2','e01418a3-d7eb-448d-8a1d-9c482990fb45','fd53835f-8adc-4332-9675-9225dde50eee','c88b335f-0edb-4359-9f0e-ed3e41c135a9','1ca6aeef-ca86-4006-8e7f-9c30a846fa44','d1241a90-d6be-41cf-bc3a-0e70d3e7753f','0e8141fb-7cf1-4b72-a43e-e22f9a0bb087','431e77e4-059c-4159-9827-995b426ef671','b8191d9f-f149-4649-88fa-da5c454439e6','994e95d2-7243-4545-bee4-be9dc5a78f58','25192014-8c94-4646-b348-bc138f289d24','5e84b834-0fb4-4ad4-8fcd-2a2dce8d913f','1a356363-9f26-4958-b4a1-5e3a6e32d08f','3b5b7448-3497-48f7-9869-7e4b9c495140','1035105e-2e8a-495c-863d-a1eeb2b28d38','71e9e0c5-50c3-41d0-bc33-6b197c083dc1','dadd1dae-354a-4e35-8af5-93c2733b6673','b5f6c23c-d3e0-41ae-968c-c3bbee34b738','9167b3aa-d85b-4ad5-af82-aa511d6e13c1','a2429ab4-7fb6-466e-95f1-25f4313f44ac','4dccfdf1-f6a0-470b-a153-ffa6f648f821','91fac8e9-1560-40cf-8ace-1c69d952fb6a','db9d0dcd-a444-4f1e-8b2e-60a63a3374d1','3ac30f11-b1a0-48c1-9616-3a84bfdc4541','d4dcacb0-037e-4ebe-8662-550bd9bab09f','2dd478a0-c250-4c36-a6d7-0f02170edd93','23d62cde-720e-45a0-80dc-ece62fe8a79b','6e695378-4272-474e-843c-bd0dafadb5fb','30ce05f2-a117-422b-9db1-53b49d33f003','c1eb53f6-e8ec-461b-930b-50d0fc08fafb','9302bf8b-8e55-4adc-987b-07bfcb9545d8','c7607c18-f485-49c1-bead-7614f7675b80','462b230d-e73a-47f8-8636-a327ffd7af4e','c2ae1a38-3545-47d2-a39b-48b2b8846a32','309e70ca-9895-4830-831e-7b47189fc5ad','0ed28340-889f-41a3-8b47-96d565c82289','e40fe7b3-99dd-492c-9823-52ef80d6430d','247fb40d-f9fb-4c81-a48c-da761156d76d','128fd641-051d-417b-9ce6-5eca029ea2d1','6e9100fe-c71d-48f7-bde7-13fd4d174316','a763e0d3-aa72-4413-88cd-b58f59d1d542','5cd57557-0a7f-464c-a737-3e574a22fcdc','2d740061-e092-43c5-9b15-f853d25f1ec5','54bd9f7d-823a-4bb1-ab37-c593fa42ed61','76fb97ed-a42b-473c-a1fc-027e2468af2c','ced7ac28-2e6a-4465-8a9e-625670ab4739','55323f97-af53-4383-b6a2-0bb134c7a4e8','45090804-d81e-4ae3-8646-7e8605c13b7f','c9c75103-0220-4a59-8096-57ade6a91c03','25d86eec-ee3b-4683-938c-1a51e105ff89','8b609c77-7dba-4987-9c70-6b40126ba1e5','4b8ababf-d535-449b-8eaa-916cb4c74271','ea6cc9b8-3522-4aa0-9877-bd5b63d92e91','3b26b576-4814-461b-981e-b98f479dab53','aba15bcc-b237-40ae-84dd-255a4e5df669','32777c41-daca-4aba-b907-e608bce7966a','d64cfbfb-7366-4bee-8772-fa34de82d4bc','58a8bc67-bfb5-4983-b19f-5b22088a9dc5','f7f499d6-7f6c-4e69-95ca-d71fdf112412','1bcdeff3-6bb2-408e-b0b4-9cce5e3e5ebe','601db135-1a71-4ffb-b0f3-e0d2c7303cb7','fc4bdd76-7e7f-4d3b-918c-bedc9a1a4e51','93bb42cb-6cf9-495f-954c-90184c1bec26','7d92d163-160b-45fa-9ea7-a5d3e53c6eb4','fe38bc4f-3aec-43f0-a4b8-29da51bb3d3f','ba148611-7928-4b2b-a591-9191cbb0b363','cda993b2-d3a4-4bc3-a3d3-94734fdc5eac','0df8d57f-0157-4ae0-885a-9c7f57834c5e','805df1ac-18fc-40a5-9a12-6756f51fcf2d','c754ede8-c7e7-4b47-88cb-4cecd064fb34','080ad2b0-4364-4052-a15b-07bd221f6abf','c7e86b97-4987-4936-94e4-81fc0312c5c6','ce78cb29-501d-49b1-8414-f6251498dca3','8a1542df-a2b5-43fd-ac36-c2e6cf84a1a8','605d94a4-29f8-4da9-aced-83a6bbdd3713','1064be33-f0dc-45f4-80bd-05b861b1e9ab','354b98b6-3804-4dd4-83b6-64235718ac83','00b8994e-754f-41a8-bdcc-d7613a88bc0c','1d1c9eee-b84e-476f-afed-5bf4ca124a65','0eee1f82-45e8-4e06-9be7-8c9beed7d0bc','c69061c4-a914-4e6b-b48d-8bed2e9a00ac','6651c467-a2c4-4ffc-9b8f-28e699227aa6','defa2c95-1ac7-4863-b494-86589ab39378','fe409676-facc-4e39-a0ef-6ebee6abaa60','705f6a46-e19e-412e-8bdf-bebcd1b67aa3','8b693a7e-de63-472d-b571-bd6c3df47c96','40cbb4fe-43fc-438f-9ae1-58318ff1a440','a622d429-db00-4925-99b5-5a62d39ed440','e1e27195-a0da-4626-8332-95882467547a','b940a082-1efb-4ec9-bde3-4dd851a96c00','ab25bc12-04d1-4d6c-a724-a2e53496de1b','9c9570db-78f9-491e-898c-2a4fb64a5433','ba8a12c1-0bf1-4c79-af0e-64353e650818','ed6acb4e-be58-4536-9522-3d897eb19ec4','4c055b33-966b-4bcf-8fea-c537219c43df','e328c68c-36f8-4518-88b1-b91e692a8432','3bc9fe64-82de-43c9-866a-14697d27101e','69a03dfb-4b97-495a-9e48-ab6cf5ef6ad5'}}),'92921',struct('BlockId','01f22f4b-6e24-4088-a5f1-2f36f2b9e2d3','SignalIds',{{'53ca05e3-9731-4f4a-8cdd-0f1937e4e7e9','9f9e8808-7f98-4a4b-bf14-9a7145728ce6','f54ae71f-9e8b-4b6c-8eea-9983ededdb22','2fd0085a-b7d0-4ec4-9e7f-36db35712486','1d7b09f8-1e81-40bf-a417-dd63c4998356','78b3f90c-de19-450b-9caa-4f8c8c164b1c','3608bdb8-911c-4ab3-9a9d-37769e1dde4a','fd166d4a-241e-4f74-913a-30a8b0fa4015','e0cf4520-9965-475d-b149-4aa5db4c721a','b30fb91b-d056-40c3-b335-d9c0fd56e001','6a5f827d-2ff5-431c-bd12-921c7afc1b21','fee74444-d8e8-45ec-b62a-5fed8bca4dd3','89d91d18-cb6d-45a5-bd38-163652f833a5','324211fc-f604-494a-bbf8-51e05583da4c','9e22aa07-a035-49fe-92a9-2c6d331da650','37ac9124-bad1-4f96-859a-3d7c4c2d26d7','276947aa-f54c-4f37-bb98-1f5926d03c2f','56e619e1-414b-4fcf-9dde-3fa79bcae4f0','946ef8bd-4767-46de-a87f-4cbd09323be9','d2043996-b496-480a-ab8a-78a7b4ac0cf4','27abb0f0-4523-4786-8486-6e82d9c24a60','5a662e81-82ff-4260-a25a-ab47e0151bb2','543cc627-7fd0-4544-a7ee-951a14aeed15','fe10dc10-882d-424c-9725-783731f5e974','25a215e3-1ac4-4d7b-a2a9-86b28d91bb89','2bf23347-477f-4f1e-a5d6-520b47f0bab3','db462e6c-768c-42f0-a44c-89f649570b02','366cca5b-5193-49e6-9376-169206ac9353','fe81c863-cb9f-4014-b168-a96d9ea111dc','c06798d7-c97f-4175-a44a-cfc61221cf4f','36e41669-6ab9-4757-9a49-4ad9030b78e1','6ae2d8e3-ae24-4f66-895e-50156a7f00a0','7ca11891-0d72-484e-a2bd-2a22e9dd0486','4f0179c6-c3f4-4108-a3d4-fcd8c59b8d68','3317a0c1-8eb3-4564-b3e5-2a1f67eb9ce6','acd8a3a2-5082-476a-a057-e8342edfea73','0f99ac7f-474b-4f93-9e2a-18d8d6e0a2f7','ed037e56-e86a-4cb5-b0dd-1afd7d0cdc0b','e51c4e5d-52b9-4ba3-858d-8ccb1ed7b833','b102886b-794e-4f9e-8d82-cf9a855382d8','9ac2a337-debf-4080-8557-b89f9504fc31'}}),'94738',struct('BlockId','bcf3b81c-74dd-45df-83eb-246bf1986e5b','SignalIds',{{'df4c9189-aad0-47af-adf9-452f98c57b31','590484b6-080e-4efb-ac1c-229f01eeeca2','6c31bfa5-0aeb-4eac-8963-270cccc0c2d7','5d56885d-f8a4-4ee4-b27f-0c2d3ee21fbc','5ee8659b-4f86-4877-ad6b-d7985f9a954b','5766d64e-9371-4170-8911-2778a90268a1','ca1e598c-d3c3-421e-9ae7-e7185f2a09d3','18fd676d-98a4-45b4-b1d7-9d0dddbc5e6f','5fed29b2-e1d1-413a-a8ac-edff34823113','279023a8-7daa-4d97-b9e1-4a91dad2ee5e','cf1bf694-ae18-42fa-a463-b9dc6cafc69e','32f22328-8598-4806-87e2-5e23a0c26b38','d9c23c5e-7a50-46d5-a10e-63ab1b9fc3b5','cf79ee48-71f6-4fd0-8aef-9c9bc30a4e49','611bb3a5-99ac-46c3-8b8b-53585c164246','d4d01821-99a2-4800-9374-6d86adaee4f2','773a5d70-a4f2-4240-9854-c19ab4783338','36678538-4ce8-44f9-9a3f-03d3e9efb7d3','ff0c1d1c-6e4d-4843-b338-e274e9a45ea7','fccb9dd1-5cda-4fe6-98ad-c7d4fc6f6931','30094c6d-d28b-4ad1-b945-e3ec2bbb07e8','fd218d85-a724-4108-b9aa-9a62089b89af','31fb8c44-bb36-419b-9e97-03acaff2a29c','a78c2e56-f9ea-44d1-b5a5-eb44b54675bd','82bf71ac-a176-45b6-9db1-c74f24b49a0b','44157694-ff9e-47f3-8066-6bd1e0cc2fce','893b8782-7964-4c73-81ba-5eb32773f42d','d274718c-9e26-4b13-ae78-5a9d797416c4','f6cb9ef7-9823-4ce2-9c69-15ccc098452a','0a99d19b-e178-42ce-b1dd-cb3f737a3d84','0d302e1f-b775-45d3-b6c8-d5c622d2f19c','c39d27b2-dc5a-4618-9837-71f8924ef39a','762f9018-3929-47c8-99b4-a7a3b2c20982'}}),'94769',struct('BlockId','ab122073-fe81-4e3c-a510-f985427cc27c','SignalIds',{{'5ef45bc3-f82f-4f11-8293-37f21f3ed968','ada81622-287d-4c74-9c00-6556f221b335','5e588d7d-6005-4734-bf0e-fe75e130e906','479383e5-dd07-4660-a182-a5d6f9c4f86f','0dc36b3e-fc07-4ded-b905-8f085d96a787','7352a0aa-a73f-4a8b-a120-1075c01938c5','b3f3e0a1-baf8-4c8e-a86c-29d225bc0e37','50d9c351-1646-431c-8cc1-f926b0084f1a','65bc14d4-7425-4c94-8508-c951edafa4db','11fd3803-ebfc-4b14-a576-ba1381606d34','3f23f25c-0dc5-4753-a10d-882186805523'}}),'95726',struct('BlockId','ef0b5d28-b6d4-4eaf-949d-d6dedf719559','SignalIds',{{'ee15b610-82c6-43bf-9a8c-0e7a9659ccea','3b41ead2-8f03-45d4-b3a2-152baba76f1c','04424910-0e7e-4b8a-bfb7-18efea10e449','d3e92efb-eafc-4308-a397-493fc39ce811','878e6af1-c668-4ab0-8e4c-5c6032b55278'}}),'95727',struct('BlockId','b2b56e4c-9e5c-48f2-8bbe-9899bbf5491a','SignalIds',{{'4e2474d8-d594-488d-9a95-ac26de9b628b'}}),'97162',struct('BlockId','609081e0-941c-41af-a124-0ef5d7529c4e','SignalIds',{{'7a0f8b5e-91b5-4be5-aa3e-8b6fa3ad27d1','46832e0a-dcde-4f52-aad9-ee2d5b2f815f','bfa458bb-0f77-4e22-9fd1-ceaff99b329a','ac728005-1b3c-4171-959f-ae8eff693e6b','008a89bc-e3d6-404d-8ad8-0ede00b346c6','21c71be8-3a66-4a2c-95b9-571df8448d55','201d8bfd-af86-4d0a-bcf2-2be355973df6','17b8c076-2f41-4633-b3f4-ebc4292cdb2d','ab00a850-8ce7-4b74-9f89-de7c76bd9fd2','240f9350-204b-43d3-8912-096b8d4fb3f9','cb628a66-37e2-44dc-ae8d-af5a0f7c0f4a','6af2e867-4ffc-447d-ba29-ba8626120048','9fcbe341-bbba-4ceb-b6e8-1ea49d1f1c20','a24cecca-e5e9-47ca-8406-22f227da4bb4','664c1055-c028-4f6c-a847-16dc729d939b','94775a18-8b75-4854-8d5a-a4dd0e581b4a','232f361b-601e-4443-b8a3-d4bc6ac96435','1fe87f67-5efa-4bdd-9d59-3c81b1c88557','81f862d0-8470-4c56-9e69-bc32aa30d43b','e1a68ded-277f-4555-a456-1524c13163e5','eab70a40-031e-4639-a10d-e5d41cb3f774','f526a80f-9956-4640-ab3a-89d2045f0162','edbb942e-05fc-4847-8de1-9a53f76b57c3','fa5191a1-3a1e-4763-8ee5-164c10c89699','50910d49-eab0-43e8-a422-548b52d3ac7c','0663fc9f-f5a9-4bfb-ae5e-87e83d32350b','eee09491-0338-41a4-874f-f2316d53c699','6f8a9a16-516f-452f-b2c6-592de3d56c59','d4fab639-aa70-4ab6-9a17-13486f62d987','8d916867-5d55-43ca-9700-dd7feeb9bc6e','eeb9a4a4-84f7-47c1-9ce7-0ef2f39b74ee','730cd9b7-4ed1-47c8-abb4-845d6e05153b','3a8d6f03-c7e0-4aec-b7ea-561ca6594a58','25840a63-a918-49a5-a812-8a1a8028e971','aef27282-f49b-416e-827e-cdd345ba9667','24938d64-a0e0-4af1-a018-252efc3ebd59','e37b8316-1f35-4643-89ab-21172ceb4edf','b22000d8-6743-4f74-a74f-a3205d460f56','071f6833-b20c-4d46-b3e4-10e823412cbb','ec3e142e-8960-4688-a09d-a55ea4e32adc','ad9531d8-6532-493d-beff-fe127dba79c1','d835263a-ecfa-4975-9fdb-449f341a58cb','eef83801-769d-4b17-8c33-06ecd7e9531f','5d0189f2-7d3e-4f08-8fe0-161cf62f662c','d2f707ad-9b49-432d-acdc-bfb37fb60912','1a39fb43-09e9-4f77-8799-5ac95783bd7a','c7276a0a-abe3-464f-bf0f-2f48a797c1e4','bd5870c5-724f-4d37-8fd7-060d6b5b46de','d639d805-c587-4e89-b332-581ad6e75f23','6efa384c-85a9-4595-b0be-cf78e9440493','53d8dcd7-0a8b-41a1-a4d7-7828db180377','9e7caebc-7806-4f8f-b588-3fafd79f3b79','2e9b888e-502d-4f3f-9192-523b6326006c','12683d1d-dbf1-47f0-883d-2f89e9585a50','0247e252-86ee-4c9b-924e-349beb4cec5d','dc694a7e-2623-4887-bd95-05da09f2976d','ebdd29c2-8c6b-4b33-8057-4a6975ea33fe','858e3f46-3ea8-485c-b4ce-1dbd84f5f4b5','bd26857f-1a73-40c8-81ea-009552807393','a67ed66b-0df4-4077-bdec-79f7b0742a37','41ba233e-5517-4492-8c6f-88d14ae87849','e89fef81-5e13-4cdd-8565-e3a4bc554c6a','79d59ed1-5a59-4091-a0a9-961027512cb9','3157c6c1-20b0-4cae-80e5-07c8fe13cb5a','96edf60c-decf-4636-b100-d32d9156fdc0','0186c05c-0b8a-45e7-acad-09290f940f36','8d0919bc-d469-4ad3-8876-2215fa1e3c58','94796f50-aca0-481f-b09f-bcd3b61dacf6','0211f4a6-eb10-4ff2-9ded-efe2f54bbcba','3fc8fd11-180d-4279-a4d1-d315f519dde3','95a29aa1-566b-46d4-92af-bb59b0582c30','74c5ffe1-f404-42ea-bd01-db28b37aef92','7582e1a1-8611-4d3c-b4a0-d1ba90126ba8','a38867d5-0379-4628-b738-91d324b276cb','1aeab194-b8fa-40b5-9dd6-7e24b15055ed','e65d4b7f-5403-4cfc-8754-8de4db2dfc3b','ceafec07-8674-4c62-89be-392175838a4f','571a7066-71e3-419d-b801-ed3605b6a94d','a339d5bc-4bac-4202-9add-1e8b4b128418','38834dd4-1316-404a-b5fb-2b6d10676a60','28b836e1-ae50-43fc-84d6-d9ce7b6871d9','7e48a4f9-6a73-4625-9ca2-29b40c8ff1d9','a2bc4953-5b0e-4e1f-b774-6d10007aa0a6','f286eacb-0890-4462-b3f9-5db0fafdecf3','86954f5f-41ea-4f72-bccd-7539044883f7','da475526-0c4c-47fd-9fc8-9468cf6b7138','eaf5dcf1-085a-4450-95d8-e0e1b31b251b','8df4d6d9-a5f5-4230-9551-006ec052d287','a6905aa2-b44b-4297-9a6d-b056c9f0f561','7c2775f6-bb4c-43c9-a1c8-611712bdfe50','f8aac724-2f6b-4507-96c6-fe2b499ca7af','c6c5d193-f81c-4525-a928-e534762a4996','1b3b3208-9784-425a-91f4-316eb01c5c0e','120ab8db-7f87-4a6d-80f3-9796dc49379f','6d4e0623-c660-4980-bc46-d841b5f15fbd','196c7c87-e6e8-439d-9c9e-2d0be2a1badc','914fd7ff-ce5e-454f-a0dc-6be5016f04e5','8fef58bc-aa80-45b7-99ac-679676dedd7e','dc22e312-d229-40ff-8255-43c4024e57f2','ea3a9df2-9771-44f4-bd80-87ab18d08c8f','d45e7130-805a-4cda-94b6-fcfd560accf8','332ff65e-4f46-4811-9c0c-aa49297458b8'}}),'97187',struct('BlockId','28a1268d-6eb1-4b71-b208-78f973de8d60','SignalIds',{{'585913a2-9f2a-482f-a871-6411ccfb653d'}}),'97198',struct('BlockId','d5a98707-e9c4-4286-94a2-1770c80d7f4f','SignalIds',{{'c855aa43-135d-4843-9f79-db840653e8fd','54417ce3-4c9d-44b2-a33a-25590b836b81','47cdef3c-44d5-42c9-abab-8063e32dbde2','c6425e0d-8cb7-4b97-9fbe-624d35a3e47c','77d2dc99-15fb-4ca0-8459-b10db5f54984','b06d46da-0afe-4348-9620-4a48ae4589bd','99f6435f-1975-4fbd-bd5f-98da826c52d2','e20ae6f0-ed78-4f04-81af-c59b4fe103ab','bb3ddaaf-07fc-4bde-931b-8b2831ae140f','369e9b5a-187f-4111-aa6d-64fcaeeff6b6','0600b854-4b29-4c2c-b5c2-771f8ef656ef','3d8d12ec-590a-4d9a-88fa-80749b59276c','a3bfa13b-5373-4658-bc35-8787c30741b4','b6e39718-75c0-406a-a8f9-b4ed2f932d63','3ae9b18c-9a42-4f93-bd17-c5884e555cba','4407ef51-ef66-4e3f-8e23-bf2f84b36441','80162738-9f36-41d3-bbbc-cd6f71812cfb','145ed585-4889-4f43-a872-6ebb3f7d528f','14ea400c-c0bd-4096-a660-ed8b908b94a1','e52b016b-0789-4cda-8e41-4c5419829fcc','d084e8ea-b9fd-47a7-a81b-404462515d73','14127863-cd8a-4aa2-ae63-f72ff16a2976','4d6dd348-42d5-4e2f-9857-af5495f942fc','9e1ffb98-cd10-47c7-bfa0-c7f82980d00f','ee3cfac1-8666-4d88-af2f-dae314b9dab0','32809660-4ebf-40a4-8fac-00ba1a8694bf','9df86f16-1321-405e-9e8f-6b65c0a77fa6','bd514d21-f259-4ce2-a044-75cb8241019b','4846c61f-afc7-4cd4-9014-9664af955811','386dabd0-67fa-4157-877a-5d180a615039','49f7453b-7d25-4dfc-a6e3-96b47f9572de','b88020d8-7bff-4d0e-bdbf-e55a3db9d2bf','f1b13c7c-ecc6-411d-82d9-5440c55df978','13a9fac6-3b2e-4e20-bb2d-49a8badf1a80','26f9ad9c-eaa6-4a90-a5c3-39f447a9ac78','0af830f9-f5e6-454f-91de-cd60639fa1e7','0560ab11-f83f-45da-9f12-4a6919fd4ced','29d2492e-438e-48be-9926-d533d6feb313','872e73e5-2920-470b-9957-414be0968712','e5f43741-853f-41ce-8e42-68a48f704f7a','43f3f7f5-28a7-4c90-a4f2-0b63d3a25f7d','a968688d-5a25-4c23-a524-134b79f7ae05','675b099e-8b6a-41f9-b872-a4bbd499150b','2ef6222d-d808-4404-8286-93450e58a407','6d426830-ae0e-4b9d-8b8e-c7a48734a28b','9d5335f9-6bfb-4110-bc63-fbe87897593b','b9f0f5a5-b551-4e47-927a-8ede67aa92d5','9afcb1de-463d-4956-bd81-daaadeee848f','22d4c151-a8b7-4096-be9d-b0fdf8528350','edfca5ed-cefb-4e7a-b682-09011c6dd0a2','27e13cb0-125d-429b-bbfa-79cf555714a8','b14b42fc-9505-403b-91f6-3fc60f9419f1','f11f7922-4891-4d2c-b4eb-aab8199e3756','1a5d8126-688f-4f87-92ea-4dfc2f81fe73','07a9e82a-eb3f-4b00-8031-1d46832aaf29','fda4505e-cb50-48ca-bcfe-4ac1460b16e2','3b2e4117-90d3-4408-94cc-bf1633040885','b0df4232-7da3-42ab-9f51-717797e8d978','89c96393-e15a-4f8c-a0bb-5addec976af0','ce89c7d6-af94-4858-9886-ba85618ff3d0','97b14e89-7e16-45b0-abcf-7b63079a139d','2959c2fd-b9c4-43c8-ae3c-0bf737823b3d','7b7f07f8-d0af-4756-8660-6fcbc2323be3','44f08197-78c1-4d08-b16b-972ccb00d32c','47ccc443-dbc0-4163-b94e-3023e1cc90f1','fee7ad07-4aad-4075-899a-d709b7f73b9f','b80ed905-e196-4089-9d38-a63c4fc3e0ff','eb35c15b-9175-47d7-a1f2-71b557a9f887','6ee26301-5de0-4a4c-876e-bac75a633ad9','e386771c-ac00-4ed2-a2fd-067c02672470','37b5cf25-dfb5-4e8f-8246-fceff19a7fd3','2b936f37-24dc-43ac-84d4-c56aa3fe720e','3931ff07-50bc-4616-823f-daba0e6bf238','3ed67b90-0b05-4a41-804c-27b0d840a85c','c1b8f6b0-29a9-4807-9733-a3d0e1039b03','067383c7-cf9d-42c8-a878-9e46b76d93a9','71f564a2-ab04-47b7-8890-1fd2a41ba090','8314a54e-ae40-44d8-bd1e-e3d36f768aa9','ba08720f-0ff3-454a-a0d8-77c8e3624210','65821741-3b91-4356-ae05-456002bb6637','013b88d3-b79b-4d63-a4ba-78498664be62','11e467c6-4f8f-40a1-bb47-6f5534593064','86b552e3-fb0d-42e3-ada8-6fb503052d11','306eb17a-03b2-4afe-8c47-fa019acc3e5b','5f9aacc0-8a99-400c-8122-8554c024806a','1c4ec95f-4377-4e8d-81c8-17e0409e5374','d5f1f4b0-a4ec-4d78-9136-f7381469164d','1932bda8-ec34-4aeb-8f11-f5cdfad08262','ce1a3840-3719-44c6-a444-2d6cf192911e','c028750a-bb52-4abf-932d-7b5a6a5342d9','87183d5b-ae04-4daf-85e4-c88dec1a53fd','8009f076-f77f-41fe-9ff8-e2e1c0c42177','5940b7e9-f37d-4acc-ac5a-f3f10831f659','1561e29a-0bae-47e8-bccd-698a30165295','74a6ff88-a32f-4536-99a7-5c33638ce392','afdefe1a-e3a3-42d4-8967-c18a8b333b14','241b2513-728f-477b-8232-42d66631417b','28b79b5a-055a-4112-bd05-df066b9a7adf','fc21657c-150a-4547-8e02-1f2f56db70b4','9574e010-78dd-4311-a59e-625492259326','b264e420-53d2-42f7-bc0a-3d486e1f3dcf','b1a0c23e-c8e3-4cf7-9b86-eac31ff31471'}}),'97223',struct('BlockId','2bb0817e-a54b-4064-8246-157ce30e8a45','SignalIds',{{'7c35180c-1def-4620-8cfc-ba0748efa5e5'}}),'97304',struct('BlockId','4118e63b-9826-405a-808d-6a2815e4502d','SignalIds',{{'01b3e1a7-f378-401f-8832-c17bbb23d801','8bb1a5ae-2220-4e72-911e-1bf42e58e4cb','dc537a66-3ee7-4b74-a769-466a6749f5f3','cc345bca-7163-4f98-8c36-d8b285b2316f','72bbf11b-86b8-413d-a3c6-b15ad8f593fa','09d8c20e-ec8b-4845-87b9-7498aee8976b','6f95cbe8-f55d-4f50-9a94-a1486b31b339','e42558b7-a07a-4146-9aaf-d538d4bcc547','a567dfdb-8fcf-4ff9-a1d2-e4b8ea8e87b0','a4a04237-9ad9-472b-9cc0-cba6eccda89e','d21b2fec-157e-4546-99aa-20a49f5b2123','cf30603d-a017-4758-b4ef-acc10542d365','f97d1c5c-89fc-42d1-b443-04b1f4566020','e5ae5f93-2521-445d-a42f-5357582259bf','1b59a933-7082-4e42-b5fb-636e4d03095e','2f90ca23-1adb-46b2-86d7-31ad12da6482','0f36c745-20f7-4ef9-9082-da06e169bfa1','061d2dc9-9131-4b99-b48a-9b0ff8d8b97c','28be56c8-312f-4e5d-b18e-1edfd44a6e2d','0e79623d-4bcf-4cbc-8070-38f639d67d18','908c7efd-3bd6-4f85-a3b6-9d52056e9c78','1cca5fa1-9e04-4d62-9101-d6ee7080ce3e','a775926e-0f86-4205-af19-7b70071a253d','19793d7c-79d9-44b8-b460-0f82d260e67f','9ca958bc-1b2b-4afc-b1ae-7d8be721e757','93e3fff1-70a8-4a0d-9417-b9de293bd010','ba446519-3a3b-49ac-89b8-b12cdaca3106','b73d54a4-a414-4181-944e-1eb485d8283c','89d5975a-ae08-413c-887f-694367b6d4b7','3175ec4d-6a41-4088-a19c-d2366275cf89','03dd4b3b-b690-4de4-8e85-f63146e35258','60627bdd-944c-4e63-8d05-4ea0006561b9','7cfda0de-925d-402d-9482-3f6fb5c606f2','240cbb01-d769-4a55-9c48-191c9f95868d','6832e2d2-1db0-4b5b-acef-28d647aab0f2','677c103b-6c9f-4bdb-bfc7-6fa9b6622754','cae61037-28de-4d53-8c0c-8a4e07abc496','1e5e87e4-d961-4212-b768-b5a8cdee5839','d5531e03-5688-4968-aa6f-7cc3599e3350','92e24c3d-ceb9-4877-95bb-ac81a5f8d155','6a1b7d30-ea42-4d8f-b0ec-1e21fc93c1cc','4559e5c9-5dc5-4cfe-b9b4-35e2b3daf863','c80a97dd-3775-4c55-94e6-856feacce23c','1f4b3783-ec57-48d5-bda0-a9f90bd3245e','9163066f-f49a-42a1-9a3d-15ea6dfa20f7','b291e216-46de-48e3-bdce-9d5f83f81ce6','7d72d178-26c6-464b-baa5-cdcc786b292a','b93ddeeb-1b31-48e9-b7ef-934d2a9e5c49','ab219c3c-0350-4a60-97ea-db06c4fee33e','6e3b383b-48b4-49c5-8c97-d9f877d2d3cc','7b66c355-0d89-468d-896b-3bb056f5e6b0','3b02ee0a-f6e7-4055-8a74-f81765a62fa6','98edbac0-0bc0-4275-b67e-d83d083685de','f12b0a52-09d5-4ab5-95d4-376bf9cdb91f','58e7d122-3c14-4ec9-be76-5a19bed4fc74','545ced7a-c299-4d81-a823-688beb87c278','8eb9c465-bca1-4103-bc99-d8a256cc79de','13a7d792-0e73-4cb9-8b76-7c831f116066','505c70cf-0ebc-4438-af82-c82737fb82b1','36cd3976-7cae-46c2-bc66-0783780c46f4','44ad4cb4-78fc-4870-a22a-c5737ca7506e','0f308031-0ae5-47ed-a451-2b0a8e74e6f2','69f4f3f7-67b9-42dc-bc25-a8b39ba3090d','080e6084-e7a7-4dd4-8b1c-1c43e9dcd6ba','74a9494f-9873-4c2c-ae76-8a0f74db06d3','ccfa1334-ed0a-46c5-b27b-0d24b3fe104c','02647cfd-7651-4591-82c0-c306a45d9954','bf5909b8-e47a-488a-97ac-8a8bb4162d68','1b52b0ef-86a9-4dcb-8cfe-32aac3b81ff3','3598f962-26f7-411e-8435-40818213f22b','1e0211c5-e0e3-470b-b0ee-33e8bcc4d108','5c746092-0c30-4e69-b43c-c92dfadd0b45','d778509b-398e-4732-8971-0ff5cebf9cf4','04576cc4-8882-4415-afa3-aeedc508a3be','c024dd67-34b1-45e3-a631-5b7bbf918376','11631a09-793b-4867-be22-79d9d65612c5','a3357929-da2a-43be-aedf-f6305debcea6','de752852-aa1c-48f2-8ef2-374d2db6bf7f','b12e6e17-85ea-4152-b69d-d16c6eb749a6','374358cb-0fa7-4c8e-92e9-037c0bb44a3c','1804bd15-cbb0-4ab3-beb3-6ef8ee465187','91472f63-d464-4e24-b37e-63823e391a72','373b3a93-b019-47b7-baeb-06c0a5a55f6c','814253fb-3bd6-4d1a-a9a5-a3f852134056','3b484bf5-91e1-4a0d-a7fa-cc4fb327c5c5','ab27b948-cf6e-4c05-947d-dfb2c65438d1','2f1b953e-1e5e-4065-9a7d-c6a7bad72005','a9f5e343-41f1-47a8-9445-7de5b8319862','0b7abe1e-ae09-4c9b-b38f-26afcca63e63','120ec359-a99a-45a5-8978-ec6ad16a0a24','a1386bd1-b3cd-4f88-82fa-66a9c6dc047d','27ff8947-825f-4a8d-b1c9-e78d91e1fc65','e484b846-ac39-427a-9333-a5dd0679e88a','a023f569-8a9b-422d-8e35-98d8b20c49a0','c6fde034-a3b0-4ecb-bb08-4786cdc61482','1ff15978-77f0-4230-8db7-739deffe4e18','2dc576c2-15f5-4b47-9974-0fc4caecf4ae','3c460159-3a51-4504-a157-b91f565eb795','5d8de635-6c66-4c6f-a0e5-69443bd37ffc','9f232409-b5b7-42be-b408-d2f2a0fdf988','0d56aaad-3931-43d6-9944-cd7d8d94e774','7ae3225f-bf53-445a-8835-56fb9d6975de'}}),'97309',struct('BlockId','c5b8f01c-70df-4224-b497-d544796a9d10','SignalIds',{{'42317a15-fedb-4030-9b34-a5b724ca26dd'}}),'97340',struct('BlockId','8b0a5312-a67c-48a9-b34f-1d6be82c8843','SignalIds',{{'f4db5faf-fb61-4c6f-b640-80cc192d1c8e','0a8a547f-22d8-4376-a9b2-5714083fb1f0','1208775c-8773-472a-bbc7-698634299448','ca05a6e5-cf91-4f1d-bc4d-28b1eef3c49d','d8eea1a8-aa7a-4d6b-8051-6bd9b610858c','5c7a2e4f-ace6-4026-a188-f979e1be3eec','bdfdada9-9c4c-477f-911c-c65d9e1ff339','2a208145-772f-47ee-9a7b-1aac75928245','0241cae5-c55a-4a65-bb99-da8f2c93baa4','4eb98ae0-8f8d-460c-87e0-ed84f1337715','a415dc3f-993e-4c04-8f62-408ce761464b','9ea75a97-370b-4a3b-9631-8371a94bc6e1','bab598bf-ac29-4c30-89d8-a221a5aa8c31','1aa88398-2c2d-4566-91b1-886bf2739ca2','435cceb2-096f-461a-97e2-2803eba8e13b','bfe550e3-05f8-43e0-92e9-29a659165fe0','575066b2-5f9d-4f7a-aafe-06d054514401','1708d4a7-b108-4092-a880-4a9233a5db3e','73bfa96d-f7ac-49ea-ae1e-07195bde5abb','74affeca-f459-4b5f-86d0-0c77c6a80cbb','bc634706-744e-481b-b24b-00ee508eb29b','740ee232-137b-42f6-a63b-d6fc7bc48afd','12569f31-0a11-4715-ae9a-329e667c8980','e6c015f0-2974-4f95-a10c-da91412374fd','4387b9aa-8d23-4a34-abe7-732fb690422b','053a1b06-d267-4261-ab75-6cddd42f835a','7ec7c7a3-3230-4240-8e12-f8259b3e50f5','4e427f28-e16d-409f-8c34-1cf947def933','4334d358-33b7-41ad-b6c7-bbbe6a15cd96','641298f3-8099-4649-a67d-48c86f0109c3','fece37c9-e9c1-41bc-9561-ca5167e3760b','c3eb5f33-0244-41d6-b000-ef71fdcec568','0423900d-d6a2-47b1-a914-20055e321f8b','2a8324e7-3ea8-48b0-92e5-d055fbeb7eab','6642d8fc-9171-4ea0-b94c-c96c126fc14d','3576bc2a-e5e0-49ad-81cc-7ebab95dd16d','d2b19811-e4b0-41bb-8d49-39b3e6b99fb0','915508e0-5c5d-44f1-9d3d-642b8c880c17','d8b08ebe-0925-4d0b-87db-03c30dda66b9','f4818373-bf5d-4163-89c7-b21ae55be742','96242654-5563-4c8e-b566-d07fbfac1306','23f357d1-3449-47e0-94f4-b286c13fb786','1ba80edb-a9cb-474d-a9e6-e513b0603c58','310de9ef-30f4-4123-ad2c-6c3e2bb8cdb8','20562b24-0576-4fc7-b017-69f3f3ccc63b','798f6ac9-f091-40c9-989f-56db13ad6a47','6ec9516c-85ea-45e9-8ab4-0093f3a91e2f','9df7552a-31cf-485e-921b-df523f724704','ec138bc5-e3eb-4cf4-87d2-e7579a9f6251','af8cb284-e6c3-47ca-b8b1-40c443f57341','64a642ba-e69e-4880-922c-edf34f504555','171efce3-6c24-4374-80ff-f06938082a4f','ceb2b419-1ef8-41f7-bb11-9d18df5d57c7','b8697e03-5a59-4bf1-aad7-541e0428d259','362a533c-6a8a-4b17-bc3f-ff9cfc142db3','82f7ee3c-0c78-4ac5-9a90-504c6e1c5f61','a3088f2d-b3a0-45c0-8664-b7c71dc4cd0b','a5de082b-ecad-4b6b-ad31-be924d507c77','7598d421-a0de-4f2f-ae81-e6ad1d58678f','24ec6dbf-6a7a-43fe-bde7-da8e87280e0f','46d535a0-a696-47b9-b3fb-1c245866e275','66d80951-c89d-4662-a7c8-904a0ad9de4f','74d4644c-6531-47cd-8e38-a372987bc87e','9b85a97d-7784-4d81-93b2-842cfc9a913f','1ab7e146-7e4b-4998-b71a-3d7a9edc6f17','f0c364af-fa8a-4c8d-8510-3d1ad58b3dee','3edcede7-5fb6-40ae-bb74-45748a2f8b04','ebbfa0b3-96d6-436f-83eb-7df4fa5f1753','31c0be34-4583-4914-bbf5-fd00b1eff51f','37146b77-3cf6-41e0-9f22-ebc5150e8b55','3c486663-aff8-471a-816b-32755038f8f1','27b815e5-a0ce-4c30-bd2b-26d85581817d','f7166b7a-6973-4b39-a16b-b8fbe3fe9cc1','feea72b2-2773-43a7-99af-916ac0b76199','eccd43b9-5fe5-4f61-9037-958e696fe794','89d86823-deea-4f9f-8fa8-aeb5a954e9e2','c116d586-a9df-4d63-a2b5-7e5c433d34c9','867b7238-5ae5-4938-a9cd-68a740cc4e21','b9c6a7e6-8024-4711-afbe-1f7024b054c4','08ff8eb0-eef2-4cd6-ad6e-24cfede8dc88','0c7c8510-5563-4676-8959-769a06cacb80','3ed829cf-810e-453b-9dcb-e522b81344b9','4759b5fd-55fa-4029-8b2b-8ea57498efe7','3a2cf3e9-867c-4245-aa08-7da53a1cddf0','05aae4f7-de30-4e26-96a9-a4f1229cc9ba','498ef53f-2fe5-4b37-8cce-a347fe2f7864','193065b8-1e38-4271-8a34-6162173ab439','e87822bd-65e9-475a-aab3-039336777ec6','a8177ff6-52df-4029-aaff-fb67f98b7c63','3f2bc1d0-9331-4d92-9e4d-7c4cdc2c3d27','22121808-fc8f-4e33-a24d-5cc22ca05efa','4faa7336-d281-484e-ae56-18def0883cac','e204e675-27e4-448f-99f0-12aa4c9f43d1','ac3856d2-afc3-4a11-b9ee-a103cba9d318','54bf5ada-91b3-4715-b3d7-7280f1698d9e','f868dc83-b00a-4e3b-ac80-5cbf1894bbd4','8bb4a648-1d86-4380-970a-d73ab9d8a0e2','bff3fa35-78e8-46f9-af03-f4eb9ffe08c5','88948313-4a10-4073-847e-eeca1014f4fd','07021bee-bc6c-4722-8770-202430afa4ff','29edcd57-f9a1-48b4-a543-d113eaf6794e','9f9f5584-5b25-413c-aaa9-bdc9a63feda1'}}),'97345',struct('BlockId','e0f8d838-16b6-419d-bd34-87d4e2e4bbee','SignalIds',{{'bd79ff19-7d83-4483-bee1-28b1bd8e11f7'}})}  OrderedModelArguments=off  Creator=GW00133806  LastModifiedBy=Cheng
settings OptimizationCC: BlockReduction=off  ConditionallyExecuteInputs=off  DefaultParameterBehavior=Inlined  OptimizeBlockIOStorage=off  BufferReuse=off  EnhancedBackFolding=on  OptimizeBlockOrder=speed  DifferentSizesBufferReuse=on
settings DebuggingCC: UnderspecifiedInitializationDetection=Classic  MergeDetectMultiDrivingBlocksExec=none  TasksWithSamePriorityMsg=none  ParameterTunabilityLossMsg=error
settings HardwareCC: ProdBitPerPointer=32  ProdBitPerSizeT=32  ProdBitPerPtrDiffT=32  ProdLargestAtomicInteger=Integer  ProdWordSize=32  ProdHWDeviceType=Custom Processor->Custom
settings ModelReferenceCC: EnableParallelModelReferenceBuilds=on  ParallelModelReferenceMATLABWorkerInit=Copy Base Workspace  ModelReferenceNumInstancesAllowed=Single  PropagateSignalLabelsOutOfModel=off
settings SFSimCC: SimParseCustomCode=off  MATLABDynamicMemAlloc=off
settings SFSimCC: SimUserIncludeDirs=|
  | .\McuEQ4Parse\src
  | .\RoadFusion_L3\src
settings RTWCC: Description=dSPACE Run-Time Target (for VEOS on Windows and ConfigurationDesk)  SystemTargetFile=dsrt.tlc  GenCodeOnly=on  MakeCommand=make_dsrt  TemplateMakefile=dsrt_default_tmf  RTWVerbose=off
settings RTWCC: CustomInclude=|
  | .\McuEQ4Parse\src
  | .\RoadFusion_L3\src
settings CodeAppCC: ForceParamTrailComments=on  MaxIdLength=128  OperatorAnnotations=on
settings STFCustomTargetCC: TargetLangStandard=C99 (ISO)  ParMdlRefBuildCompliant=on  ConcurrentExecutionCompliant=off  CPPClassGenCompliant=off  GRTInterface=off  SystemTargetFile=dsrt.tlc
settings GRTTargetCC: CompOptLevelCompliant=off  ConcurrentExecutionCompliant=off  CombineOutputUpdateFcns=off  MatFileLogging=off  CPPClassGenCompliant=off  UseToolchainInfoCompliant=off  GenerateASAP2=on

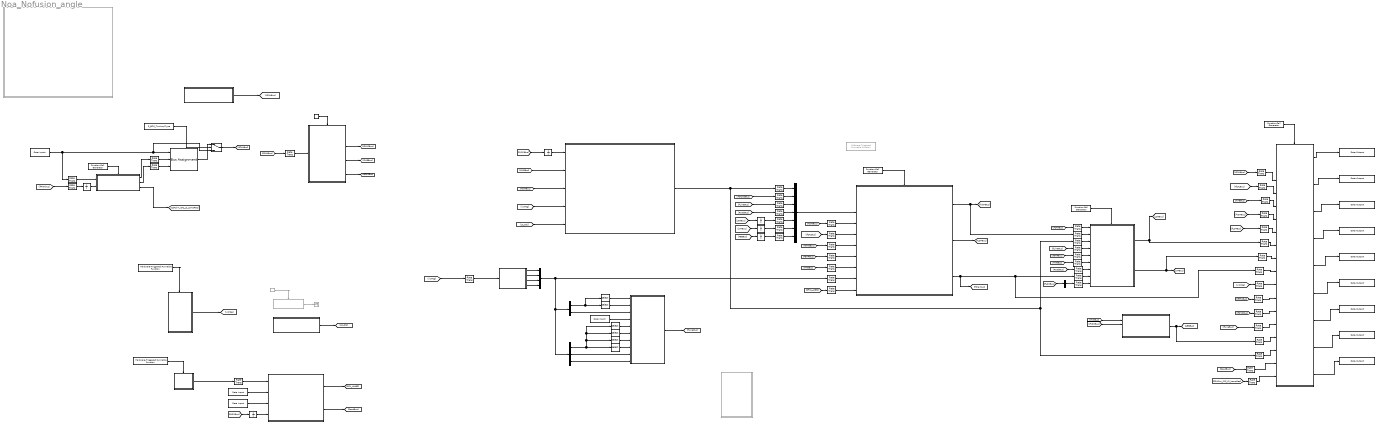
== system Noa_Nofusion_angle ==
  note: UDPReceive
  ACC_FD1 : dsmpblib/Data Outport  Priority=-10000
      settings: SourceProductName=dSPACE Model Interface Blockset
  ACC_FD2 : dsmpblib/Data Outport  Priority=-10000
      settings: SourceProductName=dSPACE Model Interface Blockset
  ACC_FD4 : dsmpblib/Data Outport  Priority=-10000
      settings: SourceProductName=dSPACE Model Interface Blockset
  Bus Assignment : BusAssignment  AssignedSignals=CSA_NODE.CSA1_MSG.LTurnLmpSwtSts,CSA_NODE.CSA1_MSG.RTurnLmpSwtSts
  Bus Creator : BusCreator  Inputs=7
  Bus Creator1 : BusCreator  Inputs=4
  Bus Selector : BusSelector  OutputSignals=EQ4_LH.EQ4_LH_ELEM,EQ4_LH.EQ4_LH_HDR
  Bus Selector1 : BusSelector  OutputSignals=LSM_HWA.RoadWidth
  Bus Selector2 : BusSelector  OutputSignals=EQ4_LA.EQ4_LA_ELEM,EQ4_LA.EQ4_LA_HDR,EQ4_LRE.EQ4_LRE_ELEM
  CAL : Subsystem
  CR_RSDS_Input : Subsystem
  Chassis1 : Subsystem
  Common : Subsystem  Tag=<DSModel=3_'Fusion'>
      settings: AttributesFormatString=<DSModel='Fusion'>
  Constant : Constant  Value=P_BCM_TurnLmpType
  Control1 : Subsystem
  Data Inport2 : dsmpblib/Data Inport  Priority=10000
      settings: SourceProductName=dSPACE Model Interface Blockset
  Data Inport7 : dsmpblib/Data Inport  Priority=10000
      settings: SourceProductName=dSPACE Model Interface Blockset
  EQ4_Lane_Pack1 : Subsystem
  Function-Call Generator{1,3..5} (4 alike) : simulink/Ports & Subsystems/Function-Call Generator  sample_time=0.02  numberOfIterations=1  DisallowWideOutput=off
  Function-Call Generator2 : simulink/Ports & Subsystems/Function-Call Generator  sample_time=0.1  numberOfIterations=1  DisallowWideOutput=off
  Function-Call Generator6 : simulink/Ports & Subsystems/Function-Call Generator  Commented=on  sample_time=0.1  numberOfIterations=1  DisallowWideOutput=off
  IDC_L3_FD1_MSG : dsmpblib/Data Outport  Priority=-10000
      settings: SourceProductName=dSPACE Model Interface Blockset
  IFC_FD{1..3,5..6} (5 alike) : dsmpblib/Data Outport  Priority=-10000
      settings: SourceProductName=dSPACE Model Interface Blockset
  IfRFM_LANES_In : dsmpblib/Data Inport  Priority=10000
      settings: SourceProductName=dSPACE Model Interface Blockset
  LPV : Subsystem
  Rate Transition{1..46} (46 alike) : RateTransition  Integrity=off  Deterministic=off
  Selector1 : Selector  InputPortWidth=4  IndexOptions=Index vector (dialog)  Indices=1  OutputSizes=1
  Selector2 : Selector  InputPortWidth=4  IndexOptions=Index vector (dialog)  Indices=2  OutputSizes=1
  Selector3 : Selector  InputPortWidth=4  IndexOptions=Index vector (dialog)  Indices=3  OutputSizes=1
  Selector4 : Selector  InputPortWidth=2  IndexOptions=Index vector (dialog)  Indices=1  OutputSizes=1
  Selector5 : Selector  InputPortWidth=2  IndexOptions=Index vector (dialog)  Indices=2  OutputSizes=1
  Selector6 : Selector  InputPortWidth=4  IndexOptions=Index vector (dialog)  Indices=4  OutputSizes=1
  SensorDia : Subsystem  Commented=on
  SimBCM : Subsystem
  Software-Triggered Runnable Function1 : dsmpblib/Software-Triggered Runnable Function  Commented=on
      settings: SourceProductName=dSPACE Model Interface Blockset
  Subsystem1 : Subsystem
  Subsystem3 : Subsystem
  Subsystem4 : Subsystem
  Subsystem5 : Subsystem  Commented=on
  Switch : Switch  Criteria=u2 ~= 0
  TOS : Subsystem
  TOS2 : Subsystem  Commented=on
  Terminator : Terminator  Commented=on
  UDP Receive (3)\Data Received : dsmpblib/Hardware-Triggered Runnable Function
      settings: SourceProductName=dSPACE Model Interface Blockset
  UDP Receive 2\Data Received : dsmpblib/Hardware-Triggered Runnable Function
      settings: SourceProductName=dSPACE Model Interface Blockset
  UDP_Received : Subsystem
  Unit Delay{,1..5} (6 alike) : UnitDelay  SampleTime=-1  HasFrameUpgradeWarning=on
  aeb : Subsystem  Tag=<DSModel=2_'Osm'>
      settings: AttributesFormatString=<DSModel='Osm'>
  ifLaneBus_out_In : dsmpblib/Data Inport  Priority=10000
      settings: SourceProductName=dSPACE Model Interface Blockset
  wires:
  [RoadBus] -> Rate Transition14/1  "roadbus"
  [RoadBus] -> Rate Transition38/1
  [IfCANBus] -> Rate Transition19/1
  [LATBus] -> Unit Delay1/1
  [IfVIEBus] -> aeb/2(IfVIEBus)
  Unit Delay3/1 -> Rate Transition39/1  "aebbus"
  Control1/1(IfLONBus) -> [LONBus], Rate Transition8/1
  [AEBBus] -> Unit Delay3/1
  Rate Transition18/1 -> Bus Creator/5  "lonbus"
  [IfEHRBus] -> Rate Transition36/1
  Control1/2(IfLATBus) -> Rate Transition7/1, [LATBus]
  [IfVIEBus] -> Rate Transition37/1
  [IfLineBus] -> Rate Transition35/1
  [LONBus] -> Unit Delay2/1
  aeb/1(IfAEBSBus) -> Rate Transition43/1, [AEBBus]
  Rate Transition20/1 -> Bus Creator/6  "latbus"
  [visMsg] -> Rate Transition16/1
  ifLaneBus_out_In/1 -> Subsystem4/4(lanebus)  "lanebus"
  TOS/1(IfTOSBus) -> Rate Transition10/1, Rate Transition44/1, Rate Transition34/1
  [ifVSMBus] -> Unit Delay/1
  [IfLineBus] -> Rate Transition13/1  "lanebus"
  [ifObjectBus] -> Rate Transition12/1
  [ifVSMBus] -> aeb/3(IfVSMBus)
  UDP Receive 2\Data Received/1 -> UDP_Received/Trigger
  UDP_Received/1(visMsg) -> [visMsg]
  Rate Transition16/1 -> Chassis1/11(IfVEQ4Bus)
  Unit Delay/1 -> TOS/1(IfStateMBus)
  [IfVIEBus] -> TOS/2(IfVIEBus)
  [IfCANBus] -> TOS/3(IfVCAN)
  EQ4_Lane_Pack1/2(EQ4_LA) -> Bus Creator1/2  "EQ4_LA"
  EQ4_Lane_Pack1/3(EQ4_LH) -> Bus Creator1/3  "EQ4_LH"
  EQ4_Lane_Pack1/4(EQ4_LRE) -> Bus Creator1/4  "EQ4_LRE"
  [visMsg] -> TOS/4(VisMsg)
  Bus Creator/1 -> LPV/3(IfALLBus)
  Rate Transition22/1 -> LPV/4(IfCANBus)
  Rate Transition23/1 -> LPV/6(IfDMSBus)
  [IfCANBus] -> Rate Transition22/1
  Rate Transition29/1 -> LPV/7(IfEHRBus)
  [IfDMSBus] -> Rate Transition23/1
  Rate Transition30/1 -> LPV/8(IfVIEBus)
  [IfVIEBus] -> Rate Transition30/1
  [IfEHRBus] -> Rate Transition29/1
  Rate Transition31/1 -> EQ4_Lane_Pack1/1(In1)  "visMsg"
  Rate Transition32/1 -> LPV/9(IfEQ4Bus)
  Function-Call Generator4/1 -> LPV/Trigger
  Function-Call Generator5/1 -> Control1/Trigger
  Rate Transition19/1 -> Control1/1(IfVCANBus)
  Rate Transition33/1 -> Control1/2(IfVSMBus)
  Rate Transition34/1 -> Control1/3(IfTOSBus)
  Rate Transition35/1 -> Control1/4(IfRFMBus)
  Rate Transition36/1 -> Control1/5(IfEHRBus)
  Rate Transition37/1 -> Control1/6(IfVIEBus)
  Rate Transition38/1 -> Control1/7(IfRoadBus)
  [visMsg] -> Rate Transition31/1
  LPV/2(IfLSMBus) -> [IfLSMBus]
  LPV/1(IfVSMBus) -> Rate Transition33/1, [ifVSMBus]
  Rate Transition10/1 -> Bus Creator/1
  Rate Transition12/1 -> Bus Creator/2
  Rate Transition13/1 -> Bus Creator/3  "lanebus"
  Rate Transition14/1 -> Bus Creator/4  "roadbus"
  Unit Delay2/1 -> Rate Transition18/1  "lonbus"
  Unit Delay1/1 -> Rate Transition20/1  "latbus"
  Rate Transition39/1 -> Bus Creator/7  "aebbus"
  [IfLineBus] -> Rate Transition1/1  "lanebus"
  Rate Transition1/1 -> Chassis1/14(LaneBus)  "lanebus"
  [IfCANBus] -> Rate Transition42/1
  CAL/1(IfCALBus) -> [IfCALBus]
  [IfCALBus] -> Rate Transition5/1
  Rate Transition5/1 -> LPV/5(IfCALBus)
  [IfCALBus] -> Rate Transition41/1
  [IfVIEBus] -> Rate Transition40/1
  [IfLSMBus] -> Rate Transition17/1
  [IfEHRBus] -> Rate Transition6/1
  [IfDMSBus] -> Rate Transition4/1
  Rate Transition6/1 -> Chassis1/12(IfEHRBus)
  Rate Transition4/1 -> Chassis1/13(IfDMSBus)
  [RoadBus] -> Rate Transition45/1  "roadbus"
  [ifVSMBus] -> Rate Transition26/1
  Rate Transition7/1 -> Chassis1/9(IfLatCtrlBus)
  Rate Transition8/1 -> Chassis1/8(IfLonCtrlBus)
  Rate Transition17/1 -> Chassis1/7(IfLSMBus)
  Rate Transition26/1 -> Chassis1/6(IfVSMBus)
  Rate Transition40/1 -> Chassis1/5(IfVIEBus)
  Rate Transition41/1 -> Chassis1/4(IfCALBus)
  Rate Transition42/1 -> Chassis1/3(IfVCANBus)
  Rate Transition43/1 -> Chassis1/15(IfAEBBus)  "lanebus"
  Rate Transition44/1 -> Chassis1/16(IfOSMBus)  "lanebus"
  Rate Transition45/1 -> Chassis1/17(RoadBus)  "lanebus"
  Function-Call Generator1/1 -> Chassis1/Trigger
  Function-Call Generator3/1 -> Common/Trigger
  [IfCANBus] -> Rate Transition3/1
  Common/2(IfDMSBus) -> [IfDMSBus]
  Common/4(IfEHRBus) -> [IfEHRBus]
  Common/3(IfVIEBus) -> [IfVIEBus]
  Rate Transition3/1 -> Common/1(IfCANBus)  "lonbus"
  LPV/3(IfPlanbus) -> [ifPlanbus], Rate Transition15/1, Rate Transition9/1
  Rate Transition9/1 -> Control1/8(IfPlanbus)
  [RFM_LANES] -> Rate Transition11/1
  Rate Transition11/1 -> LPV/10(RFM_LANES)
  EQ4_Lane_Pack1/1(EQ4_LAP) -> Bus Creator1/1  "EQ4_LAP"
  Chassis1/8(ACC_FD3) -> ACC_FD4/1
  Chassis1/1(IFC_FD1) -> IFC_FD1/1
  Chassis1/2(IFC_FD2) -> IFC_FD2/1
  Chassis1/3(IFC_FD3) -> IFC_FD3/1
  Chassis1/4(IFC_FD5) -> IFC_FD5/1
  Chassis1/5(IFC_FD6) -> IFC_FD6/1
  Chassis1/6(ACC_FD1) -> ACC_FD1/1
  Chassis1/7(ACC_FD2) -> ACC_FD2/1
  Rate Transition15/1 -> Chassis1/10(IfPlanbus)
  Rate Transition21/1 -> Subsystem1/1(l3_RFMResult)  "lonbus"
  IfRFM_LANES_In/1 -> Subsystem1/3(lane)
  Data Inport2/1 -> Subsystem1/2(road)
  Subsystem1/1(IfRFM_LANES_In) -> [RFM_LANES]
  Subsystem1/2(roadbus) -> [RoadBus]  "roadbus"
  Subsystem3/1(Out2) -> Rate Transition21/1
  UDP Receive (3)\Data Received/1 -> Subsystem3/Trigger
  CR_RSDS_Input/1(LC_Obj) -> [LC_Obj]
  [LC_Obj] -> TOS/5(LC_Obj)
  Selector4/1 -> Subsystem4/1(EQ4_LH_ELEM_0)
  Selector5/1 -> Subsystem4/2(EQ4_LH_ELEM_1)
  Bus Selector/1 -> Selector5/1, Selector4/1  "<EQ4_LH_ELEM>"
  Bus Selector/2 -> Subsystem4/3(LH_HDR)  "<EQ4_LH_HDR>"
  Subsystem4/1(Out1) -> [IfLineBus]
  [IfLSMBus] -> Bus Selector1/1
  Rate Transition24/1 -> Control1/9(roadwidth)
  Bus Selector1/1 -> Rate Transition24/1  "<RoadWidth>"
  Selector6/1 -> Subsystem4/8(EQ4_LA_ELEM_3)
  Selector3/1 -> Subsystem4/7(EQ4_LA_ELEM_2)
  Bus Selector2/3 -> Subsystem4/10(In10)  "<EQ4_LRE_ELEM>"
  Bus Selector2/1 -> Selector2/1, Selector1/1, Selector3/1, Selector6/1  "<EQ4_LA_ELEM>"
  Bus Selector2/2 -> Subsystem4/9(LA_HDR)  "<EQ4_LA_HDR>"
  Selector2/1 -> Subsystem4/6(EQ4_LA_ELEM_1)
  Bus Creator1/1 -> Bus Selector2/1, Bus Selector/1, Rate Transition32/1
  Selector1/1 -> Subsystem4/5(EQ4_LA_ELEM_0)
  Chassis1/9(IDC_L3_FD1) -> IDC_L3_FD1_MSG/1
  [IfLSMBus] -> Unit Delay4/1
  Unit Delay4/1 -> Subsystem1/4(LSMback)
  SimBCM/3(CSASim_IDC_L2_LampReq) -> [CSASim_IDC_L2_LampReq]
  [ifPlanbus] -> Rate Transition2/1
  Data Inport7/1 -> Switch/3, Bus Assignment/1, Rate Transition27/1
  Unit Delay5/1 -> SimBCM/2(PLAN_ALC_DECS)
  Rate Transition2/1 -> Unit Delay5/1
  Rate Transition46/1 -> Bus Assignment/3
  Rate Transition28/1 -> Bus Assignment/2
  [CSASim_IDC_L2_LampReq] -> Rate Transition25/1
  Rate Transition25/1 -> Chassis1/18(CSASim_IDC_L2_LampReq)  "lanebus"
  Function-Call Generator2/1 -> SimBCM/Trigger
  Rate Transition27/1 -> SimBCM/1(VCAN)
  SimBCM/1(LTurnLmpSwtSts) -> Rate Transition28/1
  SimBCM/2(RTurnLmpSwtSts) -> Rate Transition46/1
  Switch/1 -> [IfCANBus]
  Bus Assignment/1 -> Switch/1
  Constant/1 -> Switch/2
  SensorDia/1(Source_Dia_CRsts) -> Terminator/1
  Function-Call Generator6/1 -> SensorDia/Trigger
